simulink model "ScaraRobotApresentacao2023"  (R2024a)
(part 9 of 10)

et510 = dQ1.*dQ3.*m6.*t2.*t6.*t8.*t10.*t11.*t17.*-2.0-dQ1.*dQ3.*m6.*t3.*t6.*t7.*t10.*t11.*t17.*2.0+dQ1.*dQ2.*m6.*t2.*t6.*t8.*t10.*t11.*t20.*2.0+dQ1.*dQ2.*m6.*t3.*t6.*t7.*t10.*t11.*t20.*2.0-dQ1.*dQ6.*m6.*t2.*t6.*t8.*t9.*t11.*t17.*2.0-dQ1.*dQ6.*m6.*t3.*t6.*t7.*t9.*t11.*t17.*2.0+dQ1.*dQ3.*m6.*t2.*t6.*t8.*t10.*t11.*t20.*2.0+dQ1.*dQ3.*m6.*t3.*t6.*t7.*t10.*t11.*t20.*2.0-dQ2.*dQ3.*m6.*t4.*t6.*t9.*t10.*t11.*t17.*2.0+dQ1.*dQ6.*m6.*t2.*t6.*t8.*t9.*t11.*t20.*2.0+dQ1.*dQ6.*m6.*t3.*t6.*t7.*t9.*t11.*t20.*2.0+dQ2.*dQ3.*m6.*t4.*t6.*t9.*t10.*t11.*t20.*2.0+dQ1.*dQ4.*m6.*t2.*t3.*t5.*t10.*t17.*t36.*2.0-dQ1.*dQ4.*m6.*t2.*t3.*t5.*t10.*t20.*t36.*2.0-dQ1.*dQ6.*m6.*t2.*t4.*t5.*t8.*t20.*t36.*2.0-dQ1.*dQ6.*m6.*t3.*t4.*t5.*t7.*t20.*t36.*2.0-dQ1.*dQ4.*m6.*t5.*t7.*t8.*t10.*t17.*t36.*2.0;
et511 = dQ1.*dQ4.*m6.*t5.*t7.*t8.*t10.*t20.*t36.*2.0-dQ1.*dQ2.*m6.*t2.*t3.*t9.*t17.*t35.*t36.*2.0-dQ1.*dQ3.*m6.*t2.*t3.*t9.*t17.*t35.*t36.*2.0+dQ1.*dQ2.*m6.*t2.*t3.*t9.*t20.*t35.*t36.*2.0+dQ1.*dQ3.*m6.*t2.*t3.*t9.*t20.*t35.*t36.*2.0-dQ1.*dQ4.*m6.*t2.*t4.*t8.*t20.*t35.*t36.*2.0-dQ1.*dQ4.*m6.*t3.*t4.*t7.*t20.*t35.*t36.*2.0+dQ1.*dQ2.*m6.*t7.*t8.*t9.*t17.*t35.*t36.*2.0+dQ1.*dQ3.*m6.*t7.*t8.*t9.*t17.*t35.*t36.*2.0-dQ1.*dQ2.*m6.*t7.*t8.*t9.*t20.*t35.*t36.*2.0-dQ1.*dQ3.*m6.*t7.*t8.*t9.*t20.*t35.*t36.*2.0+Lx3.*Lxcm5.*dQ1.*dQ2.*m5.*t2.*t8.*t9.*t10.*2.0+Lx3.*Lxcm5.*dQ1.*dQ2.*m5.*t3.*t7.*t9.*t10.*2.0+Lx3.*Lxcm5.*dQ1.*dQ3.*m5.*t2.*t8.*t9.*t10.*2.0+Lx3.*Lxcm5.*dQ1.*dQ3.*m5.*t3.*t7.*t9.*t10.*2.0+Lx2.*Lxcm6.*dQ1.*dQ2.*m6.*t6.*t7.*t9.*t10.*2.0-Lx2.*Lycm6.*dQ1.*dQ2.*m6.*t7.*t9.*t10.*t11.*2.0;
et512 = Lxcm5.*Lycm5.*dQ1.*dQ4.*m5.*t2.*t5.*t8.*t9.*-2.0-Lxcm5.*Lycm5.*dQ1.*dQ4.*m5.*t3.*t5.*t7.*t9.*2.0+Lxcm6.*Lycm6.*dQ1.*dQ4.*m6.*t2.*t5.*t8.*t9.*2.0+Lxcm6.*Lycm6.*dQ1.*dQ4.*m6.*t3.*t5.*t7.*t9.*2.0+Lxcm6.*Lycm6.*dQ2.*dQ3.*m6.*t5.*t6.*t10.*t11.*4.0+Lxcm6.*Lycm6.*dQ2.*dQ6.*m6.*t5.*t6.*t9.*t11.*4.0+Lxcm6.*Lycm6.*dQ3.*dQ6.*m6.*t5.*t6.*t9.*t11.*4.0+Lxcm5.*Lycm5.*dQ1.*dQ2.*m5.*t2.*t8.*t10.*t34.*2.0+Lxcm5.*Lycm5.*dQ1.*dQ2.*m5.*t3.*t7.*t10.*t34.*2.0+Lxcm5.*Lycm5.*dQ1.*dQ3.*m5.*t2.*t8.*t10.*t34.*2.0+Lxcm5.*Lycm5.*dQ1.*dQ3.*m5.*t3.*t7.*t10.*t34.*2.0-Lxcm6.*Lycm6.*dQ1.*dQ2.*m6.*t2.*t8.*t10.*t34.*2.0-Lxcm6.*Lycm6.*dQ1.*dQ2.*m6.*t3.*t7.*t10.*t34.*2.0-Lxcm6.*Lycm6.*dQ1.*dQ3.*m6.*t2.*t8.*t10.*t34.*2.0-Lxcm6.*Lycm6.*dQ1.*dQ3.*m6.*t3.*t7.*t10.*t34.*2.0-Lxcm6.*Lycm6.*dQ1.*dQ2.*m6.*t2.*t8.*t10.*t36.*4.0-Lxcm6.*Lycm6.*dQ1.*dQ2.*m6.*t3.*t7.*t10.*t36.*4.0;
et513 = Lxcm6.*Lycm6.*dQ1.*dQ3.*m6.*t2.*t8.*t10.*t36.*-4.0-Lxcm6.*Lycm6.*dQ1.*dQ3.*m6.*t3.*t7.*t10.*t36.*4.0-Lxcm6.*Lycm6.*dQ1.*dQ6.*m6.*t2.*t8.*t9.*t36.*4.0-Lxcm6.*Lycm6.*dQ1.*dQ6.*m6.*t3.*t7.*t9.*t36.*4.0-Lxcm6.*Lycm6.*dQ2.*dQ3.*m6.*t4.*t9.*t10.*t36.*4.0+Lxcm6.*Lycm6.*dQ2.*dQ4.*m6.*t6.*t9.*t11.*t35.*4.0+Lxcm6.*Lycm6.*dQ3.*dQ4.*m6.*t6.*t9.*t11.*t35.*4.0-Lx3.*Lz5.*dQ1.*dQ2.*m6.*t2.*t5.*t8.*t9.*2.0-Lx3.*Lz5.*dQ1.*dQ2.*m6.*t3.*t5.*t7.*t9.*2.0-Lx3.*Lz5.*dQ1.*dQ3.*m6.*t2.*t5.*t8.*t9.*2.0-Lx3.*Lz5.*dQ1.*dQ3.*m6.*t3.*t5.*t7.*t9.*2.0-Lx3.*Lzcm5.*dQ1.*dQ2.*m5.*t2.*t5.*t8.*t9.*2.0-Lx3.*Lzcm5.*dQ1.*dQ2.*m5.*t3.*t5.*t7.*t9.*2.0-Lxcm6.*Lz5.*dQ1.*dQ6.*m6.*t2.*t3.*t5.*t6.*2.0-Lx3.*Lzcm5.*dQ1.*dQ3.*m5.*t2.*t5.*t8.*t9.*2.0-Lx3.*Lzcm5.*dQ1.*dQ3.*m5.*t3.*t5.*t7.*t9.*2.0;
et514 = Lxcm5.*Lz4.*dQ1.*dQ2.*m5.*t2.*t3.*t9.*t10.*-2.0-Lx3.*Lzcm6.*dQ1.*dQ2.*m6.*t2.*t5.*t8.*t9.*2.0-Lx3.*Lzcm6.*dQ1.*dQ2.*m6.*t3.*t5.*t7.*t9.*2.0-Lxcm5.*Lz4.*dQ1.*dQ3.*m5.*t2.*t3.*t9.*t10.*2.0-Lx3.*Lzcm6.*dQ1.*dQ3.*m6.*t2.*t5.*t8.*t9.*2.0-Lx3.*Lzcm6.*dQ1.*dQ3.*m6.*t3.*t5.*t7.*t9.*2.0+Lxcm6.*Lz5.*dQ1.*dQ2.*m6.*t2.*t5.*t8.*t11.*2.0+Lxcm6.*Lz5.*dQ1.*dQ2.*m6.*t3.*t5.*t7.*t11.*2.0+Lxcm6.*Lz5.*dQ1.*dQ3.*m6.*t2.*t5.*t8.*t11.*2.0+Lxcm6.*Lz5.*dQ1.*dQ3.*m6.*t3.*t5.*t7.*t11.*2.0+Lxcm6.*Lz5.*dQ1.*dQ6.*m6.*t5.*t6.*t7.*t8.*2.0+Lxcm5.*Lz4.*dQ1.*dQ2.*m5.*t7.*t8.*t9.*t10.*2.0+Lxcm6.*Lz5.*dQ2.*dQ3.*m6.*t4.*t5.*t9.*t11.*2.0+Lxcm5.*Lz4.*dQ1.*dQ3.*m5.*t7.*t8.*t9.*t10.*2.0-Lxcm6.*Lz5.*dQ2.*dQ4.*m6.*t5.*t6.*t9.*t10.*4.0-Lxcm6.*Lz5.*dQ3.*dQ4.*m6.*t5.*t6.*t9.*t10.*4.0-Lxcm6.*Lz5.*dQ1.*dQ4.*m6.*t2.*t3.*t6.*t35.*4.0;
et515 = Lxcm6.*Lz5.*dQ1.*dQ4.*m6.*t6.*t7.*t8.*t35.*4.0+Lxcm5.*Lzcm5.*dQ1.*dQ2.*m5.*t2.*t4.*t8.*t9.*2.0+Lxcm5.*Lzcm5.*dQ1.*dQ2.*m5.*t3.*t4.*t7.*t9.*2.0-Lxcm6.*Lzcm6.*dQ1.*dQ6.*m6.*t2.*t3.*t5.*t6.*2.0+Lxcm5.*Lzcm5.*dQ1.*dQ3.*m5.*t2.*t4.*t8.*t9.*2.0+Lxcm5.*Lzcm5.*dQ1.*dQ3.*m5.*t3.*t4.*t7.*t9.*2.0+Lxcm6.*Lzcm6.*dQ1.*dQ2.*m6.*t2.*t5.*t8.*t11.*2.0+Lxcm6.*Lzcm6.*dQ1.*dQ2.*m6.*t3.*t5.*t7.*t11.*2.0+Lxcm6.*Lzcm6.*dQ1.*dQ3.*m6.*t2.*t5.*t8.*t11.*2.0+Lxcm6.*Lzcm6.*dQ1.*dQ3.*m6.*t3.*t5.*t7.*t11.*2.0+Lxcm6.*Lzcm6.*dQ1.*dQ6.*m6.*t5.*t6.*t7.*t8.*2.0+Lxcm6.*Lzcm6.*dQ2.*dQ3.*m6.*t4.*t5.*t9.*t11.*2.0-Lxcm6.*Lzcm6.*dQ2.*dQ4.*m6.*t5.*t6.*t9.*t10.*4.0-Lxcm6.*Lzcm6.*dQ3.*dQ4.*m6.*t5.*t6.*t9.*t10.*4.0-Lxcm6.*Lzcm6.*dQ1.*dQ4.*m6.*t2.*t3.*t6.*t35.*4.0+Lxcm6.*Lzcm6.*dQ1.*dQ4.*m6.*t6.*t7.*t8.*t35.*4.0+Lycm6.*Lz5.*dQ1.*dQ2.*m6.*t2.*t5.*t6.*t8.*2.0;
et516 = Lycm6.*Lz5.*dQ1.*dQ2.*m6.*t3.*t5.*t6.*t7.*2.0+Lycm6.*Lz5.*dQ1.*dQ3.*m6.*t2.*t5.*t6.*t8.*2.0+Lycm6.*Lz5.*dQ1.*dQ3.*m6.*t3.*t5.*t6.*t7.*2.0+Lycm6.*Lz5.*dQ1.*dQ6.*m6.*t2.*t3.*t5.*t11.*2.0+Lycm6.*Lz5.*dQ2.*dQ3.*m6.*t4.*t5.*t6.*t9.*2.0-Lycm6.*Lz5.*dQ1.*dQ6.*m6.*t5.*t7.*t8.*t11.*2.0+Lycm6.*Lz5.*dQ2.*dQ4.*m6.*t5.*t9.*t10.*t11.*4.0+Lycm6.*Lz5.*dQ3.*dQ4.*m6.*t5.*t9.*t10.*t11.*4.0+Lycm6.*Lz5.*dQ1.*dQ4.*m6.*t2.*t3.*t11.*t35.*4.0-Lycm6.*Lz5.*dQ1.*dQ4.*m6.*t7.*t8.*t11.*t35.*4.0+Lycm6.*Lzcm6.*dQ1.*dQ2.*m6.*t2.*t5.*t6.*t8.*2.0+Lycm6.*Lzcm6.*dQ1.*dQ2.*m6.*t3.*t5.*t6.*t7.*2.0+Lycm6.*Lzcm6.*dQ1.*dQ3.*m6.*t2.*t5.*t6.*t8.*2.0+Lycm6.*Lzcm6.*dQ1.*dQ3.*m6.*t3.*t5.*t6.*t7.*2.0+Lycm6.*Lzcm6.*dQ1.*dQ6.*m6.*t2.*t3.*t5.*t11.*2.0+Lycm6.*Lzcm6.*dQ2.*dQ3.*m6.*t4.*t5.*t6.*t9.*2.0-Lycm5.*Lzcm5.*dQ1.*dQ4.*m5.*t2.*t8.*t9.*t10.*2.0;
et517 = Lycm5.*Lzcm5.*dQ1.*dQ4.*m5.*t3.*t7.*t9.*t10.*-2.0-Lycm6.*Lzcm6.*dQ1.*dQ6.*m6.*t5.*t7.*t8.*t11.*2.0+Lycm6.*Lzcm6.*dQ2.*dQ4.*m6.*t5.*t9.*t10.*t11.*4.0+Lycm6.*Lzcm6.*dQ3.*dQ4.*m6.*t5.*t9.*t10.*t11.*4.0-Lycm5.*Lzcm5.*dQ1.*dQ2.*m5.*t2.*t5.*t8.*t34.*2.0-Lycm5.*Lzcm5.*dQ1.*dQ2.*m5.*t3.*t5.*t7.*t34.*2.0-Lycm5.*Lzcm5.*dQ1.*dQ3.*m5.*t2.*t5.*t8.*t34.*2.0-Lycm5.*Lzcm5.*dQ1.*dQ3.*m5.*t3.*t5.*t7.*t34.*2.0+Lycm6.*Lzcm6.*dQ1.*dQ4.*m6.*t2.*t3.*t11.*t35.*4.0-Lycm6.*Lzcm6.*dQ1.*dQ4.*m6.*t7.*t8.*t11.*t35.*4.0+Lz4.*Lz5.*dQ1.*dQ2.*m6.*t2.*t3.*t5.*t9.*2.0+Lz4.*Lz5.*dQ1.*dQ3.*m6.*t2.*t3.*t5.*t9.*2.0-Lz4.*Lz5.*dQ1.*dQ2.*m6.*t5.*t7.*t8.*t9.*2.0-Lz4.*Lz5.*dQ1.*dQ3.*m6.*t5.*t7.*t8.*t9.*2.0+Lz4.*Lzcm5.*dQ1.*dQ2.*m5.*t2.*t3.*t5.*t9.*2.0+Lz4.*Lzcm5.*dQ1.*dQ3.*m5.*t2.*t3.*t5.*t9.*2.0+Lz4.*Lzcm6.*dQ1.*dQ2.*m6.*t2.*t3.*t5.*t9.*2.0;
et518 = Lz4.*Lzcm6.*dQ1.*dQ3.*m6.*t2.*t3.*t5.*t9.*2.0-Lz5.*Lzcm6.*dQ1.*dQ4.*m6.*t2.*t3.*t5.*t10.*4.0-Lz4.*Lzcm5.*dQ1.*dQ2.*m5.*t5.*t7.*t8.*t9.*2.0-Lz4.*Lzcm5.*dQ1.*dQ3.*m5.*t5.*t7.*t8.*t9.*2.0-Lz4.*Lzcm6.*dQ1.*dQ2.*m6.*t5.*t7.*t8.*t9.*2.0-Lz4.*Lzcm6.*dQ1.*dQ3.*m6.*t5.*t7.*t8.*t9.*2.0+Lz5.*Lzcm6.*dQ1.*dQ4.*m6.*t5.*t7.*t8.*t10.*4.0+Lz5.*Lzcm6.*dQ1.*dQ2.*m6.*t2.*t3.*t9.*t35.*4.0+Lz5.*Lzcm6.*dQ1.*dQ3.*m6.*t2.*t3.*t9.*t35.*4.0-Lz5.*Lzcm6.*dQ1.*dQ4.*m6.*t2.*t4.*t8.*t35.*4.0-Lz5.*Lzcm6.*dQ1.*dQ4.*m6.*t3.*t4.*t7.*t35.*4.0-Lz5.*Lzcm6.*dQ1.*dQ2.*m6.*t7.*t8.*t9.*t35.*4.0-Lz5.*Lzcm6.*dQ1.*dQ3.*m6.*t7.*t8.*t9.*t35.*4.0+Lx3.*Lxcm6.*dQ1.*dQ2.*m6.*t2.*t6.*t8.*t9.*t10.*2.0+Lx3.*Lxcm6.*dQ1.*dQ2.*m6.*t3.*t6.*t7.*t9.*t10.*2.0+Lx3.*Lxcm6.*dQ1.*dQ3.*m6.*t2.*t6.*t8.*t9.*t10.*2.0+Lx3.*Lxcm6.*dQ1.*dQ3.*m6.*t3.*t6.*t7.*t9.*t10.*2.0;
et519 = Lx3.*Lycm6.*dQ1.*dQ2.*m6.*t2.*t8.*t9.*t10.*t11.*-2.0-Lx3.*Lycm6.*dQ1.*dQ2.*m6.*t3.*t7.*t9.*t10.*t11.*2.0-Lx3.*Lycm6.*dQ1.*dQ3.*m6.*t2.*t8.*t9.*t10.*t11.*2.0-Lx3.*Lycm6.*dQ1.*dQ3.*m6.*t3.*t7.*t9.*t10.*t11.*2.0-Lxcm6.*Lycm6.*dQ1.*dQ2.*m6.*t2.*t3.*t6.*t9.*t11.*4.0-Lxcm6.*Lycm6.*dQ1.*dQ3.*m6.*t2.*t3.*t6.*t9.*t11.*4.0-Lxcm6.*Lycm6.*dQ1.*dQ6.*m6.*t2.*t3.*t6.*t10.*t11.*4.0+Lxcm6.*Lycm6.*dQ1.*dQ2.*m6.*t6.*t7.*t8.*t9.*t11.*4.0+Lxcm6.*Lycm6.*dQ1.*dQ3.*m6.*t6.*t7.*t8.*t9.*t11.*4.0+Lxcm6.*Lycm6.*dQ1.*dQ6.*m6.*t6.*t7.*t8.*t10.*t11.*4.0-Lxcm6.*Lycm6.*dQ1.*dQ4.*m6.*t2.*t5.*t8.*t9.*t36.*4.0-Lxcm6.*Lycm6.*dQ1.*dQ4.*m6.*t3.*t5.*t7.*t9.*t36.*4.0-Lxcm6.*Lycm6.*dQ2.*dQ3.*m6.*t5.*t6.*t10.*t11.*t34.*4.0+Lxcm6.*Lycm6.*dQ1.*dQ2.*m6.*t2.*t8.*t10.*t34.*t36.*4.0+Lxcm6.*Lycm6.*dQ1.*dQ2.*m6.*t3.*t7.*t10.*t34.*t36.*4.0;
et520 = Lxcm6.*Lycm6.*dQ1.*dQ3.*m6.*t2.*t8.*t10.*t34.*t36.*4.0+Lxcm6.*Lycm6.*dQ1.*dQ3.*m6.*t3.*t7.*t10.*t34.*t36.*4.0-Lxcm6.*Lz4.*dQ1.*dQ2.*m6.*t2.*t3.*t6.*t9.*t10.*2.0+Lxcm6.*Lz5.*dQ1.*dQ2.*m6.*t2.*t4.*t6.*t8.*t9.*2.0+Lxcm6.*Lz5.*dQ1.*dQ2.*m6.*t3.*t4.*t6.*t7.*t9.*2.0-Lxcm6.*Lz4.*dQ1.*dQ3.*m6.*t2.*t3.*t6.*t9.*t10.*2.0+Lxcm6.*Lz5.*dQ1.*dQ3.*m6.*t2.*t4.*t6.*t8.*t9.*2.0+Lxcm6.*Lz5.*dQ1.*dQ3.*m6.*t3.*t4.*t6.*t7.*t9.*2.0+Lxcm6.*Lz5.*dQ1.*dQ6.*m6.*t2.*t4.*t6.*t8.*t10.*2.0+Lxcm6.*Lz5.*dQ1.*dQ6.*m6.*t3.*t4.*t6.*t7.*t10.*2.0+Lxcm6.*Lz4.*dQ1.*dQ2.*m6.*t6.*t7.*t8.*t9.*t10.*2.0+Lxcm6.*Lz4.*dQ1.*dQ3.*m6.*t6.*t7.*t8.*t9.*t10.*2.0-Lxcm6.*Lz5.*dQ1.*dQ4.*m6.*t2.*t8.*t9.*t10.*t11.*2.0-Lxcm6.*Lz5.*dQ1.*dQ4.*m6.*t3.*t7.*t9.*t10.*t11.*2.0-Lxcm6.*Lz5.*dQ1.*dQ2.*m6.*t2.*t5.*t8.*t11.*t34.*2.0-Lxcm6.*Lz5.*dQ1.*dQ2.*m6.*t3.*t5.*t7.*t11.*t34.*2.0;
et521 = Lxcm6.*Lz5.*dQ1.*dQ3.*m6.*t2.*t5.*t8.*t11.*t34.*-2.0-Lxcm6.*Lz5.*dQ1.*dQ3.*m6.*t3.*t5.*t7.*t11.*t34.*2.0-Lxcm5.*Lzcm5.*dQ1.*dQ2.*m5.*t2.*t3.*t5.*t9.*t10.*4.0-Lxcm5.*Lzcm5.*dQ1.*dQ3.*m5.*t2.*t3.*t5.*t9.*t10.*4.0+Lxcm5.*Lzcm5.*dQ1.*dQ4.*m5.*t2.*t4.*t5.*t8.*t10.*4.0+Lxcm5.*Lzcm5.*dQ1.*dQ4.*m5.*t3.*t4.*t5.*t7.*t10.*4.0+Lxcm6.*Lzcm6.*dQ1.*dQ2.*m6.*t2.*t4.*t6.*t8.*t9.*2.0+Lxcm6.*Lzcm6.*dQ1.*dQ2.*m6.*t3.*t4.*t6.*t7.*t9.*2.0+Lxcm6.*Lzcm6.*dQ1.*dQ3.*m6.*t2.*t4.*t6.*t8.*t9.*2.0+Lxcm6.*Lzcm6.*dQ1.*dQ3.*m6.*t3.*t4.*t6.*t7.*t9.*2.0+Lxcm6.*Lzcm6.*dQ1.*dQ6.*m6.*t2.*t4.*t6.*t8.*t10.*2.0+Lxcm6.*Lzcm6.*dQ1.*dQ6.*m6.*t3.*t4.*t6.*t7.*t10.*2.0+Lxcm5.*Lzcm5.*dQ1.*dQ2.*m5.*t5.*t7.*t8.*t9.*t10.*4.0+Lxcm5.*Lzcm5.*dQ1.*dQ3.*m5.*t5.*t7.*t8.*t9.*t10.*4.0-Lxcm6.*Lzcm6.*dQ1.*dQ4.*m6.*t2.*t8.*t9.*t10.*t11.*2.0-Lxcm6.*Lzcm6.*dQ1.*dQ4.*m6.*t3.*t7.*t9.*t10.*t11.*2.0;
et522 = Lxcm5.*Lzcm5.*dQ1.*dQ2.*m5.*t2.*t4.*t8.*t9.*t35.*-4.0-Lxcm5.*Lzcm5.*dQ1.*dQ2.*m5.*t3.*t4.*t7.*t9.*t35.*4.0-Lxcm5.*Lzcm5.*dQ1.*dQ3.*m5.*t2.*t4.*t8.*t9.*t35.*4.0-Lxcm5.*Lzcm5.*dQ1.*dQ3.*m5.*t3.*t4.*t7.*t9.*t35.*4.0-Lxcm6.*Lzcm6.*dQ1.*dQ2.*m6.*t2.*t5.*t8.*t11.*t34.*2.0-Lxcm6.*Lzcm6.*dQ1.*dQ2.*m6.*t3.*t5.*t7.*t11.*t34.*2.0-Lxcm6.*Lzcm6.*dQ1.*dQ3.*m6.*t2.*t5.*t8.*t11.*t34.*2.0-Lxcm6.*Lzcm6.*dQ1.*dQ3.*m6.*t3.*t5.*t7.*t11.*t34.*2.0+Lycm6.*Lz4.*dQ1.*dQ2.*m6.*t2.*t3.*t9.*t10.*t11.*2.0-Lycm6.*Lz5.*dQ1.*dQ2.*m6.*t2.*t4.*t8.*t9.*t11.*2.0-Lycm6.*Lz5.*dQ1.*dQ2.*m6.*t3.*t4.*t7.*t9.*t11.*2.0+Lycm6.*Lz4.*dQ1.*dQ3.*m6.*t2.*t3.*t9.*t10.*t11.*2.0-Lycm6.*Lz5.*dQ1.*dQ3.*m6.*t2.*t4.*t8.*t9.*t11.*2.0-Lycm6.*Lz5.*dQ1.*dQ3.*m6.*t3.*t4.*t7.*t9.*t11.*2.0-Lycm6.*Lz5.*dQ1.*dQ4.*m6.*t2.*t6.*t8.*t9.*t10.*2.0;
et523 = Lycm6.*Lz5.*dQ1.*dQ4.*m6.*t3.*t6.*t7.*t9.*t10.*-2.0-Lycm6.*Lz5.*dQ1.*dQ6.*m6.*t2.*t4.*t8.*t10.*t11.*2.0-Lycm6.*Lz5.*dQ1.*dQ6.*m6.*t3.*t4.*t7.*t10.*t11.*2.0-Lycm6.*Lz4.*dQ1.*dQ2.*m6.*t7.*t8.*t9.*t10.*t11.*2.0-Lycm6.*Lz4.*dQ1.*dQ3.*m6.*t7.*t8.*t9.*t10.*t11.*2.0-Lycm6.*Lz5.*dQ1.*dQ2.*m6.*t2.*t5.*t6.*t8.*t34.*2.0-Lycm6.*Lz5.*dQ1.*dQ2.*m6.*t3.*t5.*t6.*t7.*t34.*2.0-Lycm6.*Lz5.*dQ1.*dQ3.*m6.*t2.*t5.*t6.*t8.*t34.*2.0-Lycm6.*Lz5.*dQ1.*dQ3.*m6.*t3.*t5.*t6.*t7.*t34.*2.0-Lycm6.*Lzcm6.*dQ1.*dQ2.*m6.*t2.*t4.*t8.*t9.*t11.*2.0-Lycm6.*Lzcm6.*dQ1.*dQ2.*m6.*t3.*t4.*t7.*t9.*t11.*2.0-Lycm6.*Lzcm6.*dQ1.*dQ3.*m6.*t2.*t4.*t8.*t9.*t11.*2.0-Lycm6.*Lzcm6.*dQ1.*dQ3.*m6.*t3.*t4.*t7.*t9.*t11.*2.0-Lycm6.*Lzcm6.*dQ1.*dQ4.*m6.*t2.*t6.*t8.*t9.*t10.*2.0-Lycm6.*Lzcm6.*dQ1.*dQ4.*m6.*t3.*t6.*t7.*t9.*t10.*2.0;
et524 = Lycm6.*Lzcm6.*dQ1.*dQ6.*m6.*t2.*t4.*t8.*t10.*t11.*-2.0-Lycm6.*Lzcm6.*dQ1.*dQ6.*m6.*t3.*t4.*t7.*t10.*t11.*2.0-Lycm6.*Lzcm6.*dQ1.*dQ2.*m6.*t2.*t5.*t6.*t8.*t34.*2.0-Lycm6.*Lzcm6.*dQ1.*dQ2.*m6.*t3.*t5.*t6.*t7.*t34.*2.0-Lycm6.*Lzcm6.*dQ1.*dQ3.*m6.*t2.*t5.*t6.*t8.*t34.*2.0-Lycm6.*Lzcm6.*dQ1.*dQ3.*m6.*t3.*t5.*t6.*t7.*t34.*2.0-Ixx6.*dQ1.*dQ2.*t2.*t4.*t5.*t8.*t9.*t10.*t36.*2.0-Ixx6.*dQ1.*dQ2.*t3.*t4.*t5.*t7.*t9.*t10.*t36.*2.0-Ixx6.*dQ1.*dQ3.*t2.*t4.*t5.*t8.*t9.*t10.*t36.*2.0-Ixx6.*dQ1.*dQ3.*t3.*t4.*t5.*t7.*t9.*t10.*t36.*2.0+Iyy6.*dQ1.*dQ2.*t2.*t4.*t5.*t8.*t9.*t10.*t36.*2.0+Iyy6.*dQ1.*dQ2.*t3.*t4.*t5.*t7.*t9.*t10.*t36.*2.0+Iyy6.*dQ1.*dQ3.*t2.*t4.*t5.*t8.*t9.*t10.*t36.*2.0+Iyy6.*dQ1.*dQ3.*t3.*t4.*t5.*t7.*t9.*t10.*t36.*2.0+dQ1.*dQ2.*m5.*t2.*t4.*t5.*t8.*t9.*t10.*t16.*2.0;
et525 = dQ1.*dQ2.*m5.*t3.*t4.*t5.*t7.*t9.*t10.*t16.*2.0+dQ1.*dQ3.*m5.*t2.*t4.*t5.*t8.*t9.*t10.*t16.*2.0+dQ1.*dQ3.*m5.*t3.*t4.*t5.*t7.*t9.*t10.*t16.*2.0+dQ1.*dQ2.*m6.*t2.*t4.*t5.*t8.*t9.*t10.*t20.*2.0+dQ1.*dQ2.*m6.*t3.*t4.*t5.*t7.*t9.*t10.*t20.*2.0+dQ1.*dQ3.*m6.*t2.*t4.*t5.*t8.*t9.*t10.*t20.*2.0+dQ1.*dQ3.*m6.*t3.*t4.*t5.*t7.*t9.*t10.*t20.*2.0-dQ1.*dQ2.*m6.*t2.*t4.*t5.*t8.*t9.*t10.*t22.*2.0-dQ1.*dQ2.*m6.*t3.*t4.*t5.*t7.*t9.*t10.*t22.*2.0-dQ1.*dQ4.*m6.*t2.*t5.*t6.*t8.*t9.*t11.*t17.*2.0-dQ1.*dQ4.*m6.*t3.*t5.*t6.*t7.*t9.*t11.*t17.*2.0-dQ1.*dQ3.*m6.*t2.*t4.*t5.*t8.*t9.*t10.*t22.*2.0-dQ1.*dQ3.*m6.*t3.*t4.*t5.*t7.*t9.*t10.*t22.*2.0-dQ1.*dQ2.*m5.*t2.*t4.*t5.*t8.*t9.*t10.*t25.*2.0-dQ1.*dQ2.*m5.*t3.*t4.*t5.*t7.*t9.*t10.*t25.*2.0;
et526 = dQ1.*dQ3.*m5.*t2.*t4.*t5.*t8.*t9.*t10.*t25.*-2.0-dQ1.*dQ3.*m5.*t3.*t4.*t5.*t7.*t9.*t10.*t25.*2.0+dQ1.*dQ4.*m6.*t2.*t5.*t6.*t8.*t9.*t11.*t20.*2.0+dQ1.*dQ4.*m6.*t3.*t5.*t6.*t7.*t9.*t11.*t20.*2.0-dQ1.*dQ2.*m6.*t2.*t4.*t5.*t8.*t9.*t10.*t26.*2.0-dQ1.*dQ2.*m6.*t3.*t4.*t5.*t7.*t9.*t10.*t26.*2.0-dQ1.*dQ3.*m6.*t2.*t4.*t5.*t8.*t9.*t10.*t26.*2.0-dQ1.*dQ3.*m6.*t3.*t4.*t5.*t7.*t9.*t10.*t26.*2.0+dQ1.*dQ2.*m6.*t2.*t6.*t8.*t10.*t11.*t17.*t34.*2.0+dQ1.*dQ2.*m6.*t3.*t6.*t7.*t10.*t11.*t17.*t34.*2.0+dQ1.*dQ3.*m6.*t2.*t6.*t8.*t10.*t11.*t17.*t34.*2.0+dQ1.*dQ3.*m6.*t3.*t6.*t7.*t10.*t11.*t17.*t34.*2.0-dQ1.*dQ2.*m6.*t2.*t6.*t8.*t10.*t11.*t20.*t34.*2.0-dQ1.*dQ2.*m6.*t3.*t6.*t7.*t10.*t11.*t20.*t34.*2.0-dQ1.*dQ3.*m6.*t2.*t6.*t8.*t10.*t11.*t20.*t34.*2.0;
et527 = dQ1.*dQ3.*m6.*t3.*t6.*t7.*t10.*t11.*t20.*t34.*-2.0-Ixy6.*dQ1.*dQ2.*t2.*t4.*t5.*t6.*t8.*t9.*t10.*t11.*2.0-Ixy6.*dQ1.*dQ2.*t3.*t4.*t5.*t6.*t7.*t9.*t10.*t11.*2.0-Ixy6.*dQ1.*dQ3.*t2.*t4.*t5.*t6.*t8.*t9.*t10.*t11.*2.0-Ixy6.*dQ1.*dQ3.*t3.*t4.*t5.*t6.*t7.*t9.*t10.*t11.*2.0-Iyx6.*dQ1.*dQ2.*t2.*t4.*t5.*t6.*t8.*t9.*t10.*t11.*2.0-Iyx6.*dQ1.*dQ2.*t3.*t4.*t5.*t6.*t7.*t9.*t10.*t11.*2.0-Iyx6.*dQ1.*dQ3.*t2.*t4.*t5.*t6.*t8.*t9.*t10.*t11.*2.0-Iyx6.*dQ1.*dQ3.*t3.*t4.*t5.*t6.*t7.*t9.*t10.*t11.*2.0+dQ1.*dQ2.*m6.*t2.*t4.*t5.*t8.*t9.*t10.*t17.*t36.*2.0+dQ1.*dQ2.*m6.*t3.*t4.*t5.*t7.*t9.*t10.*t17.*t36.*2.0+dQ1.*dQ3.*m6.*t2.*t4.*t5.*t8.*t9.*t10.*t17.*t36.*2.0+dQ1.*dQ3.*m6.*t3.*t4.*t5.*t7.*t9.*t10.*t17.*t36.*2.0-dQ1.*dQ2.*m6.*t2.*t4.*t5.*t8.*t9.*t10.*t20.*t36.*2.0;
et528 = dQ1.*dQ2.*m6.*t3.*t4.*t5.*t7.*t9.*t10.*t20.*t36.*-2.0-dQ1.*dQ3.*m6.*t2.*t4.*t5.*t8.*t9.*t10.*t20.*t36.*2.0-dQ1.*dQ3.*m6.*t3.*t4.*t5.*t7.*t9.*t10.*t20.*t36.*2.0-Lxcm6.*Lycm6.*dQ1.*dQ4.*m6.*t2.*t3.*t5.*t6.*t10.*t11.*4.0-Lxcm6.*Lycm6.*dQ1.*dQ6.*m6.*t2.*t4.*t5.*t6.*t8.*t11.*4.0-Lxcm6.*Lycm6.*dQ1.*dQ6.*m6.*t3.*t4.*t5.*t6.*t7.*t11.*4.0+Lxcm6.*Lycm6.*dQ1.*dQ4.*m6.*t5.*t6.*t7.*t8.*t10.*t11.*4.0+Lxcm6.*Lycm6.*dQ1.*dQ2.*m6.*t2.*t3.*t6.*t9.*t11.*t35.*4.0+Lxcm6.*Lycm6.*dQ1.*dQ3.*m6.*t2.*t3.*t6.*t9.*t11.*t35.*4.0-Lxcm6.*Lycm6.*dQ1.*dQ4.*m6.*t2.*t4.*t6.*t8.*t11.*t35.*4.0-Lxcm6.*Lycm6.*dQ1.*dQ4.*m6.*t3.*t4.*t6.*t7.*t11.*t35.*4.0-Lxcm6.*Lycm6.*dQ1.*dQ2.*m6.*t6.*t7.*t8.*t9.*t11.*t35.*4.0-Lxcm6.*Lycm6.*dQ1.*dQ3.*m6.*t6.*t7.*t8.*t9.*t11.*t35.*4.0-Lxcm6.*Lz5.*dQ1.*dQ2.*m6.*t2.*t3.*t5.*t6.*t9.*t10.*4.0;
et529 = Lxcm6.*Lz5.*dQ1.*dQ3.*m6.*t2.*t3.*t5.*t6.*t9.*t10.*-4.0+Lxcm6.*Lz5.*dQ1.*dQ4.*m6.*t2.*t4.*t5.*t6.*t8.*t10.*4.0+Lxcm6.*Lz5.*dQ1.*dQ4.*m6.*t3.*t4.*t5.*t6.*t7.*t10.*4.0+Lxcm6.*Lz5.*dQ1.*dQ2.*m6.*t5.*t6.*t7.*t8.*t9.*t10.*4.0+Lxcm6.*Lz5.*dQ1.*dQ3.*m6.*t5.*t6.*t7.*t8.*t9.*t10.*4.0-Lxcm6.*Lz5.*dQ1.*dQ2.*m6.*t2.*t4.*t6.*t8.*t9.*t35.*4.0-Lxcm6.*Lz5.*dQ1.*dQ2.*m6.*t3.*t4.*t6.*t7.*t9.*t35.*4.0-Lxcm6.*Lz5.*dQ1.*dQ3.*m6.*t2.*t4.*t6.*t8.*t9.*t35.*4.0-Lxcm6.*Lz5.*dQ1.*dQ3.*m6.*t3.*t4.*t6.*t7.*t9.*t35.*4.0-Lxcm6.*Lzcm6.*dQ1.*dQ2.*m6.*t2.*t3.*t5.*t6.*t9.*t10.*4.0-Lxcm6.*Lzcm6.*dQ1.*dQ3.*m6.*t2.*t3.*t5.*t6.*t9.*t10.*4.0+Lxcm6.*Lzcm6.*dQ1.*dQ4.*m6.*t2.*t4.*t5.*t6.*t8.*t10.*4.0+Lxcm6.*Lzcm6.*dQ1.*dQ4.*m6.*t3.*t4.*t5.*t6.*t7.*t10.*4.0+Lxcm6.*Lzcm6.*dQ1.*dQ2.*m6.*t5.*t6.*t7.*t8.*t9.*t10.*4.0;
et530 = Lxcm6.*Lzcm6.*dQ1.*dQ3.*m6.*t5.*t6.*t7.*t8.*t9.*t10.*4.0-Lxcm6.*Lzcm6.*dQ1.*dQ2.*m6.*t2.*t4.*t6.*t8.*t9.*t35.*4.0-Lxcm6.*Lzcm6.*dQ1.*dQ2.*m6.*t3.*t4.*t6.*t7.*t9.*t35.*4.0-Lxcm6.*Lzcm6.*dQ1.*dQ3.*m6.*t2.*t4.*t6.*t8.*t9.*t35.*4.0-Lxcm6.*Lzcm6.*dQ1.*dQ3.*m6.*t3.*t4.*t6.*t7.*t9.*t35.*4.0+Lycm6.*Lz5.*dQ1.*dQ2.*m6.*t2.*t3.*t5.*t9.*t10.*t11.*4.0+Lycm6.*Lz5.*dQ1.*dQ3.*m6.*t2.*t3.*t5.*t9.*t10.*t11.*4.0-Lycm6.*Lz5.*dQ1.*dQ4.*m6.*t2.*t4.*t5.*t8.*t10.*t11.*4.0-Lycm6.*Lz5.*dQ1.*dQ4.*m6.*t3.*t4.*t5.*t7.*t10.*t11.*4.0-Lycm6.*Lz5.*dQ1.*dQ2.*m6.*t5.*t7.*t8.*t9.*t10.*t11.*4.0-Lycm6.*Lz5.*dQ1.*dQ3.*m6.*t5.*t7.*t8.*t9.*t10.*t11.*4.0+Lycm6.*Lz5.*dQ1.*dQ2.*m6.*t2.*t4.*t8.*t9.*t11.*t35.*4.0+Lycm6.*Lz5.*dQ1.*dQ2.*m6.*t3.*t4.*t7.*t9.*t11.*t35.*4.0+Lycm6.*Lz5.*dQ1.*dQ3.*m6.*t2.*t4.*t8.*t9.*t11.*t35.*4.0;
et531 = Lycm6.*Lz5.*dQ1.*dQ3.*m6.*t3.*t4.*t7.*t9.*t11.*t35.*4.0+Lycm6.*Lzcm6.*dQ1.*dQ2.*m6.*t2.*t3.*t5.*t9.*t10.*t11.*4.0+Lycm6.*Lzcm6.*dQ1.*dQ3.*m6.*t2.*t3.*t5.*t9.*t10.*t11.*4.0-Lycm6.*Lzcm6.*dQ1.*dQ4.*m6.*t2.*t4.*t5.*t8.*t10.*t11.*4.0-Lycm6.*Lzcm6.*dQ1.*dQ4.*m6.*t3.*t4.*t5.*t7.*t10.*t11.*4.0-Lycm6.*Lzcm6.*dQ1.*dQ2.*m6.*t5.*t7.*t8.*t9.*t10.*t11.*4.0-Lycm6.*Lzcm6.*dQ1.*dQ3.*m6.*t5.*t7.*t8.*t9.*t10.*t11.*4.0+Lycm6.*Lzcm6.*dQ1.*dQ2.*m6.*t2.*t4.*t8.*t9.*t11.*t35.*4.0+Lycm6.*Lzcm6.*dQ1.*dQ2.*m6.*t3.*t4.*t7.*t9.*t11.*t35.*4.0+Lycm6.*Lzcm6.*dQ1.*dQ3.*m6.*t2.*t4.*t8.*t9.*t11.*t35.*4.0+Lycm6.*Lzcm6.*dQ1.*dQ3.*m6.*t3.*t4.*t7.*t9.*t11.*t35.*4.0-Lz5.*Lzcm6.*dQ1.*dQ2.*m6.*t2.*t4.*t5.*t8.*t9.*t10.*4.0-Lz5.*Lzcm6.*dQ1.*dQ2.*m6.*t3.*t4.*t5.*t7.*t9.*t10.*4.0-Lz5.*Lzcm6.*dQ1.*dQ3.*m6.*t2.*t4.*t5.*t8.*t9.*t10.*4.0;
et532 = Lz5.*Lzcm6.*dQ1.*dQ3.*m6.*t3.*t4.*t5.*t7.*t9.*t10.*-4.0-Lxcm6.*Lycm6.*dQ1.*dQ2.*m6.*t2.*t4.*t5.*t6.*t8.*t9.*t10.*t11.*4.0-Lxcm6.*Lycm6.*dQ1.*dQ2.*m6.*t3.*t4.*t5.*t6.*t7.*t9.*t10.*t11.*4.0-Lxcm6.*Lycm6.*dQ1.*dQ3.*m6.*t2.*t4.*t5.*t6.*t8.*t9.*t10.*t11.*4.0-Lxcm6.*Lycm6.*dQ1.*dQ3.*m6.*t3.*t4.*t5.*t6.*t7.*t9.*t10.*t11.*4.0;
et533 = t9.*t10.*t55+t9.*t10.*t56+t9.*t10.*t62+t9.*t10.*t63+t9.*t10.*t82+t9.*t10.*t83+t9.*t10.*t84+t9.*t10.*t85+t9.*t10.*t88+t9.*t10.*t89+t9.*t10.*t90+t9.*t10.*t91+t9.*t10.*t138+t9.*t10.*t139+t9.*t10.*t150+t9.*t10.*t151+t9.*t10.*t177+t9.*t10.*t178+t9.*t10.*t179+t9.*t10.*t180+t9.*t10.*t307+t9.*t10.*t308+t9.*t10.*t333+t9.*t10.*t334+t9.*t10.*t342+t9.*t10.*t343+t9.*t10.*t418+t9.*t10.*t419+t9.*t10.*t615+t9.*t10.*t616+t9.*t10.*t674+t9.*t10.*t675+t9.*t10.*t687+t9.*t10.*t688+t9.*t10.*t761+t9.*t10.*t762+t9.*t10.*t776+t9.*t10.*t777+t9.*t10.*t942+t9.*t10.*t943+t9.*t10.*t1096+t9.*t10.*t1097+t9.*t10.*t1481+t9.*t10.*t1482+t9.*t10.*t1642+t9.*t10.*t1643-t9.*t10.*t36.*t138.*2.0-t9.*t10.*t36.*t139.*2.0;
et534 = -Ixx6.*dQ4.*dQ5.*t10-Ixy6.*dQ2.*dQ5.*t4-Ixy6.*dQ3.*dQ5.*t4-Ixy6.*dQ2.*dQ3.*t34+Ixy6.*dQ2.*dQ3.*t35-Iyx6.*dQ2.*dQ5.*t4-Iyx6.*dQ3.*dQ5.*t4-Iyx6.*dQ2.*dQ3.*t34+Iyx6.*dQ2.*dQ3.*t35+Iyy6.*dQ4.*dQ5.*t10-Izz6.*dQ4.*dQ5.*t10-Ixx6.*dQ2.*dQ4.*t4.*t10+Ixx6.*dQ2.*dQ5.*t5.*t9-Ixx6.*dQ3.*dQ4.*t4.*t10+Ixx6.*dQ3.*dQ5.*t5.*t9+Ixx6.*dQ4.*dQ5.*t10.*t36.*2.0+Ixy6.*dQ1.*dQ4.*t2.*t3-Ixy6.*dQ1.*dQ4.*t7.*t8+Ixy6.*dQ2.*dQ5.*t4.*t36.*2.0+Ixy6.*dQ3.*dQ5.*t4.*t36.*2.0-Ixy6.*dQ2.*dQ3.*t34.*t35+Ixy6.*dQ2.*dQ3.*t34.*t36.*2.0-Ixy6.*dQ2.*dQ3.*t35.*t36.*2.0+Ixz6.*dQ4.*dQ5.*t5.*t6+Ixz6.*dQ2.*dQ4.*t9.*t11+Ixz6.*dQ3.*dQ4.*t9.*t11+Iyx6.*dQ1.*dQ4.*t2.*t3-Iyx6.*dQ1.*dQ4.*t7.*t8+Iyx6.*dQ2.*dQ5.*t4.*t36.*2.0;
et535 = Iyx6.*dQ3.*dQ5.*t4.*t36.*2.0-Iyx6.*dQ2.*dQ3.*t34.*t35+Iyx6.*dQ2.*dQ3.*t34.*t36.*2.0-Iyx6.*dQ2.*dQ3.*t35.*t36.*2.0+Iyy6.*dQ2.*dQ4.*t4.*t10-Iyy6.*dQ2.*dQ5.*t5.*t9+Iyy6.*dQ3.*dQ4.*t4.*t10-Iyy6.*dQ3.*dQ5.*t5.*t9-Iyy6.*dQ4.*dQ5.*t10.*t36.*2.0+Iyz6.*dQ2.*dQ4.*t6.*t9+Iyz6.*dQ3.*dQ4.*t6.*t9-Iyz6.*dQ4.*dQ5.*t5.*t11+Izx6.*dQ4.*dQ5.*t5.*t6+Izx6.*dQ2.*dQ4.*t9.*t11+Izx6.*dQ3.*dQ4.*t9.*t11+Izy6.*dQ2.*dQ4.*t6.*t9+Izy6.*dQ3.*dQ4.*t6.*t9-Izy6.*dQ4.*dQ5.*t5.*t11+Izz6.*dQ2.*dQ4.*t4.*t10+Izz6.*dQ2.*dQ5.*t5.*t9+Izz6.*dQ3.*dQ4.*t4.*t10+Izz6.*dQ3.*dQ5.*t5.*t9-dQ4.*dQ5.*m6.*t10.*t20.*2.0+t4.*t5.*t6.*t10.*t11.*t130.*2.0+t4.*t5.*t6.*t10.*t11.*t131.*2.0-t4.*t5.*t6.*t10.*t11.*t138.*2.0-t4.*t5.*t6.*t10.*t11.*t139.*2.0-Lxcm6.*Lycm6.*dQ2.*dQ5.*m6.*t4.*2.0;
et536 = Lxcm6.*Lycm6.*dQ3.*dQ5.*m6.*t4.*-2.0-Lxcm6.*Lycm6.*dQ2.*dQ3.*m6.*t34.*2.0+Lxcm6.*Lycm6.*dQ2.*dQ3.*m6.*t35.*2.0+Ixx6.*dQ1.*dQ2.*t2.*t5.*t8+Ixx6.*dQ1.*dQ2.*t3.*t5.*t7+Ixx6.*dQ1.*dQ3.*t2.*t5.*t8+Ixx6.*dQ1.*dQ3.*t3.*t5.*t7-Ixx6.*dQ1.*dQ5.*t2.*t3.*t10+Ixx6.*dQ2.*dQ3.*t4.*t5.*t9.*2.0-Ixx6.*dQ2.*dQ5.*t4.*t6.*t11.*2.0-Ixx6.*dQ3.*dQ5.*t4.*t6.*t11.*2.0+Ixx6.*dQ1.*dQ5.*t7.*t8.*t10-Ixx6.*dQ2.*dQ3.*t6.*t11.*t34.*2.0+Ixx6.*dQ2.*dQ4.*t4.*t10.*t36.*2.0+Ixx6.*dQ2.*dQ3.*t6.*t11.*t35.*2.0-Ixx6.*dQ2.*dQ5.*t5.*t9.*t36.*2.0+Ixx6.*dQ3.*dQ4.*t4.*t10.*t36.*2.0-Ixx6.*dQ3.*dQ5.*t5.*t9.*t36.*2.0-Ixy6.*dQ1.*dQ5.*t2.*t8.*t9-Ixy6.*dQ1.*dQ5.*t3.*t7.*t9+Ixy6.*dQ4.*dQ5.*t6.*t10.*t11.*2.0-Ixy6.*dQ1.*dQ4.*t2.*t3.*t35-Ixy6.*dQ1.*dQ4.*t2.*t3.*t36.*2.0+Ixy6.*dQ1.*dQ4.*t7.*t8.*t35;
et537 = Ixy6.*dQ1.*dQ4.*t7.*t8.*t36.*2.0+Ixy6.*dQ2.*dQ3.*t34.*t35.*t36.*2.0-Ixz6.*dQ2.*dQ3.*t5.*t10.*t11-Ixz6.*dQ2.*dQ4.*t9.*t11.*t35-Ixz6.*dQ3.*dQ4.*t9.*t11.*t35-Iyx6.*dQ1.*dQ5.*t2.*t8.*t9-Iyx6.*dQ1.*dQ5.*t3.*t7.*t9+Iyx6.*dQ4.*dQ5.*t6.*t10.*t11.*2.0-Iyx6.*dQ1.*dQ4.*t2.*t3.*t35-Iyx6.*dQ1.*dQ4.*t2.*t3.*t36.*2.0+Iyx6.*dQ1.*dQ4.*t7.*t8.*t35+Iyx6.*dQ1.*dQ4.*t7.*t8.*t36.*2.0+Iyx6.*dQ2.*dQ3.*t34.*t35.*t36.*2.0-Iyy6.*dQ1.*dQ2.*t2.*t5.*t8-Iyy6.*dQ1.*dQ2.*t3.*t5.*t7-Iyy6.*dQ1.*dQ3.*t2.*t5.*t8-Iyy6.*dQ1.*dQ3.*t3.*t5.*t7+Iyy6.*dQ1.*dQ5.*t2.*t3.*t10-Iyy6.*dQ2.*dQ3.*t4.*t5.*t9.*2.0+Iyy6.*dQ2.*dQ5.*t4.*t6.*t11.*2.0+Iyy6.*dQ3.*dQ5.*t4.*t6.*t11.*2.0-Iyy6.*dQ1.*dQ5.*t7.*t8.*t10+Iyy6.*dQ2.*dQ3.*t6.*t11.*t34.*2.0;
et538 = Iyy6.*dQ2.*dQ4.*t4.*t10.*t36.*-2.0-Iyy6.*dQ2.*dQ3.*t6.*t11.*t35.*2.0+Iyy6.*dQ2.*dQ5.*t5.*t9.*t36.*2.0-Iyy6.*dQ3.*dQ4.*t4.*t10.*t36.*2.0+Iyy6.*dQ3.*dQ5.*t5.*t9.*t36.*2.0-Iyz6.*dQ2.*dQ3.*t5.*t6.*t10-Iyz6.*dQ2.*dQ4.*t6.*t9.*t35-Iyz6.*dQ3.*dQ4.*t6.*t9.*t35-Izx6.*dQ2.*dQ3.*t5.*t10.*t11-Izx6.*dQ2.*dQ4.*t9.*t11.*t35-Izx6.*dQ3.*dQ4.*t9.*t11.*t35-Izy6.*dQ2.*dQ3.*t5.*t6.*t10-Izy6.*dQ2.*dQ4.*t6.*t9.*t35-Izy6.*dQ3.*dQ4.*t6.*t9.*t35-Izz6.*dQ1.*dQ2.*t2.*t5.*t8-Izz6.*dQ1.*dQ2.*t3.*t5.*t7-Izz6.*dQ1.*dQ3.*t2.*t5.*t8-Izz6.*dQ1.*dQ3.*t3.*t5.*t7-Izz6.*dQ1.*dQ5.*t2.*t3.*t10+Izz6.*dQ1.*dQ5.*t7.*t8.*t10+dQ2.*dQ4.*m6.*t4.*t10.*t17.*2.0+dQ3.*dQ4.*m6.*t4.*t10.*t17.*2.0+dQ2.*dQ5.*m6.*t5.*t9.*t20.*2.0;
et539 = dQ3.*dQ5.*m6.*t5.*t9.*t20.*2.0-dQ4.*dQ5.*m6.*t10.*t17.*t36.*2.0+dQ4.*dQ5.*m6.*t10.*t20.*t36.*2.0+Lx3.*Lxcm6.*dQ2.*dQ3.*m6.*t6.*t9.*2.0-Lx3.*Lycm6.*dQ2.*dQ3.*m6.*t9.*t11.*2.0+Lxcm6.*Lycm6.*dQ1.*dQ4.*m6.*t2.*t3.*2.0-Lxcm6.*Lycm6.*dQ1.*dQ4.*m6.*t7.*t8.*2.0+Lxcm6.*Lycm6.*dQ2.*dQ5.*m6.*t4.*t36.*4.0+Lxcm6.*Lycm6.*dQ3.*dQ5.*m6.*t4.*t36.*4.0-Lxcm6.*Lycm6.*dQ2.*dQ3.*m6.*t34.*t35.*2.0+Lxcm6.*Lycm6.*dQ2.*dQ3.*m6.*t34.*t36.*4.0-Lxcm6.*Lycm6.*dQ2.*dQ3.*m6.*t35.*t36.*4.0+Lxcm6.*Lz5.*dQ4.*dQ5.*m6.*t5.*t6.*2.0-Lxcm6.*Lz4.*dQ2.*dQ3.*m6.*t10.*t11.*2.0+Lxcm6.*Lz5.*dQ2.*dQ4.*m6.*t9.*t11.*2.0+Lxcm6.*Lz5.*dQ3.*dQ4.*m6.*t9.*t11.*2.0+Lxcm6.*Lzcm6.*dQ4.*dQ5.*m6.*t5.*t6.*2.0+Lxcm6.*Lzcm6.*dQ2.*dQ4.*m6.*t9.*t11.*2.0+Lxcm6.*Lzcm6.*dQ3.*dQ4.*m6.*t9.*t11.*2.0-Lycm6.*Lz4.*dQ2.*dQ3.*m6.*t6.*t10.*2.0+Lycm6.*Lz5.*dQ2.*dQ4.*m6.*t6.*t9.*2.0;
et540 = Lycm6.*Lz5.*dQ3.*dQ4.*m6.*t6.*t9.*2.0-Lycm6.*Lz5.*dQ4.*dQ5.*m6.*t5.*t11.*2.0+Lycm6.*Lzcm6.*dQ2.*dQ4.*m6.*t6.*t9.*2.0+Lycm6.*Lzcm6.*dQ3.*dQ4.*m6.*t6.*t9.*2.0-Lycm6.*Lzcm6.*dQ4.*dQ5.*m6.*t5.*t11.*2.0-Ixx6.*dQ1.*dQ2.*t2.*t3.*t4.*t10-Ixx6.*dQ1.*dQ3.*t2.*t3.*t4.*t10-Ixx6.*dQ1.*dQ5.*t2.*t4.*t5.*t8-Ixx6.*dQ1.*dQ5.*t3.*t4.*t5.*t7+Ixx6.*dQ1.*dQ4.*t2.*t3.*t6.*t11.*2.0+Ixx6.*dQ1.*dQ2.*t4.*t7.*t8.*t10+Ixx6.*dQ1.*dQ3.*t4.*t7.*t8.*t10-Ixx6.*dQ1.*dQ4.*t6.*t7.*t8.*t11.*2.0-Ixx6.*dQ1.*dQ2.*t2.*t5.*t8.*t34.*2.0-Ixx6.*dQ1.*dQ2.*t3.*t5.*t7.*t34.*2.0-Ixx6.*dQ1.*dQ3.*t2.*t5.*t8.*t34.*2.0-Ixx6.*dQ1.*dQ3.*t3.*t5.*t7.*t34.*2.0-Ixx6.*dQ1.*dQ2.*t2.*t5.*t8.*t36.*2.0-Ixx6.*dQ1.*dQ2.*t3.*t5.*t7.*t36.*2.0-Ixx6.*dQ1.*dQ3.*t2.*t5.*t8.*t36.*2.0;
et541 = Ixx6.*dQ1.*dQ3.*t3.*t5.*t7.*t36.*-2.0+Ixx6.*dQ1.*dQ5.*t2.*t3.*t10.*t36.*2.0-Ixx6.*dQ2.*dQ3.*t4.*t5.*t9.*t36.*4.0-Ixx6.*dQ1.*dQ5.*t7.*t8.*t10.*t36.*2.0-Ixx6.*dQ2.*dQ3.*t6.*t11.*t34.*t35.*2.0-Ixy6.*dQ1.*dQ2.*t2.*t4.*t8.*t9-Ixy6.*dQ1.*dQ2.*t3.*t4.*t7.*t9-Ixy6.*dQ1.*dQ3.*t2.*t4.*t8.*t9-Ixy6.*dQ1.*dQ3.*t3.*t4.*t7.*t9+Ixy6.*dQ2.*dQ4.*t4.*t6.*t10.*t11.*2.0-Ixy6.*dQ2.*dQ5.*t5.*t6.*t9.*t11.*2.0+Ixy6.*dQ3.*dQ4.*t4.*t6.*t10.*t11.*2.0-Ixy6.*dQ3.*dQ5.*t5.*t6.*t9.*t11.*2.0+Ixy6.*dQ1.*dQ5.*t2.*t8.*t9.*t36.*2.0+Ixy6.*dQ1.*dQ5.*t3.*t7.*t9.*t36.*2.0+Ixy6.*dQ1.*dQ4.*t2.*t3.*t35.*t36.*2.0-Ixy6.*dQ1.*dQ4.*t7.*t8.*t35.*t36.*2.0+Ixz6.*dQ1.*dQ5.*t2.*t3.*t5.*t6-Ixz6.*dQ1.*dQ4.*t2.*t4.*t8.*t11-Ixz6.*dQ1.*dQ4.*t3.*t4.*t7.*t11;
et542 = -Ixz6.*dQ1.*dQ5.*t5.*t6.*t7.*t8+Ixz6.*dQ2.*dQ3.*t4.*t6.*t9.*t10+Ixz6.*dQ2.*dQ3.*t5.*t10.*t11.*t34-Iyx6.*dQ1.*dQ2.*t2.*t4.*t8.*t9-Iyx6.*dQ1.*dQ2.*t3.*t4.*t7.*t9-Iyx6.*dQ1.*dQ3.*t2.*t4.*t8.*t9-Iyx6.*dQ1.*dQ3.*t3.*t4.*t7.*t9+Iyx6.*dQ2.*dQ4.*t4.*t6.*t10.*t11.*2.0-Iyx6.*dQ2.*dQ5.*t5.*t6.*t9.*t11.*2.0+Iyx6.*dQ3.*dQ4.*t4.*t6.*t10.*t11.*2.0-Iyx6.*dQ3.*dQ5.*t5.*t6.*t9.*t11.*2.0+Iyx6.*dQ1.*dQ5.*t2.*t8.*t9.*t36.*2.0+Iyx6.*dQ1.*dQ5.*t3.*t7.*t9.*t36.*2.0+Iyx6.*dQ1.*dQ4.*t2.*t3.*t35.*t36.*2.0-Iyx6.*dQ1.*dQ4.*t7.*t8.*t35.*t36.*2.0+Iyy6.*dQ1.*dQ2.*t2.*t3.*t4.*t10+Iyy6.*dQ1.*dQ3.*t2.*t3.*t4.*t10+Iyy6.*dQ1.*dQ5.*t2.*t4.*t5.*t8+Iyy6.*dQ1.*dQ5.*t3.*t4.*t5.*t7-Iyy6.*dQ1.*dQ4.*t2.*t3.*t6.*t11.*2.0-Iyy6.*dQ1.*dQ2.*t4.*t7.*t8.*t10;
et543 = -Iyy6.*dQ1.*dQ3.*t4.*t7.*t8.*t10+Iyy6.*dQ1.*dQ4.*t6.*t7.*t8.*t11.*2.0+Iyy6.*dQ1.*dQ2.*t2.*t5.*t8.*t34.*2.0+Iyy6.*dQ1.*dQ2.*t3.*t5.*t7.*t34.*2.0+Iyy6.*dQ1.*dQ3.*t2.*t5.*t8.*t34.*2.0+Iyy6.*dQ1.*dQ3.*t3.*t5.*t7.*t34.*2.0+Iyy6.*dQ1.*dQ2.*t2.*t5.*t8.*t36.*2.0+Iyy6.*dQ1.*dQ2.*t3.*t5.*t7.*t36.*2.0+Iyy6.*dQ1.*dQ3.*t2.*t5.*t8.*t36.*2.0+Iyy6.*dQ1.*dQ3.*t3.*t5.*t7.*t36.*2.0-Iyy6.*dQ1.*dQ5.*t2.*t3.*t10.*t36.*2.0+Iyy6.*dQ2.*dQ3.*t4.*t5.*t9.*t36.*4.0+Iyy6.*dQ1.*dQ5.*t7.*t8.*t10.*t36.*2.0+Iyy6.*dQ2.*dQ3.*t6.*t11.*t34.*t35.*2.0-Iyz6.*dQ1.*dQ4.*t2.*t4.*t6.*t8-Iyz6.*dQ1.*dQ4.*t3.*t4.*t6.*t7-Iyz6.*dQ1.*dQ5.*t2.*t3.*t5.*t11+Iyz6.*dQ1.*dQ5.*t5.*t7.*t8.*t11-Iyz6.*dQ2.*dQ3.*t4.*t9.*t10.*t11+Iyz6.*dQ2.*dQ3.*t5.*t6.*t10.*t34+Izx6.*dQ1.*dQ5.*t2.*t3.*t5.*t6;
et544 = -Izx6.*dQ1.*dQ4.*t2.*t4.*t8.*t11-Izx6.*dQ1.*dQ4.*t3.*t4.*t7.*t11-Izx6.*dQ1.*dQ5.*t5.*t6.*t7.*t8+Izx6.*dQ2.*dQ3.*t4.*t6.*t9.*t10+Izx6.*dQ2.*dQ3.*t5.*t10.*t11.*t34-Izy6.*dQ1.*dQ4.*t2.*t4.*t6.*t8-Izy6.*dQ1.*dQ4.*t3.*t4.*t6.*t7-Izy6.*dQ1.*dQ5.*t2.*t3.*t5.*t11+Izy6.*dQ1.*dQ5.*t5.*t7.*t8.*t11-Izy6.*dQ2.*dQ3.*t4.*t9.*t10.*t11+Izy6.*dQ2.*dQ3.*t5.*t6.*t10.*t34-Izz6.*dQ1.*dQ2.*t2.*t3.*t4.*t10-Izz6.*dQ1.*dQ3.*t2.*t3.*t4.*t10-Izz6.*dQ1.*dQ5.*t2.*t4.*t5.*t8-Izz6.*dQ1.*dQ5.*t3.*t4.*t5.*t7+Izz6.*dQ1.*dQ2.*t4.*t7.*t8.*t10+Izz6.*dQ1.*dQ3.*t4.*t7.*t8.*t10-dQ1.*dQ2.*m6.*t2.*t5.*t8.*t17.*2.0-dQ1.*dQ2.*m6.*t3.*t5.*t7.*t17.*2.0-dQ1.*dQ3.*m6.*t2.*t5.*t8.*t17.*2.0-dQ1.*dQ3.*m6.*t3.*t5.*t7.*t17.*2.0;
et545 = dQ2.*dQ3.*m6.*t4.*t5.*t9.*t17.*-2.0-dQ1.*dQ5.*m6.*t2.*t3.*t10.*t20.*2.0+dQ2.*dQ3.*m6.*t4.*t5.*t9.*t20.*2.0+dQ2.*dQ5.*m6.*t4.*t6.*t11.*t17.*2.0+dQ3.*dQ5.*m6.*t4.*t6.*t11.*t17.*2.0-dQ2.*dQ5.*m6.*t4.*t6.*t11.*t20.*2.0-dQ3.*dQ5.*m6.*t4.*t6.*t11.*t20.*2.0+dQ1.*dQ5.*m6.*t7.*t8.*t10.*t20.*2.0+dQ2.*dQ3.*m6.*t6.*t11.*t17.*t34.*2.0-dQ2.*dQ4.*m6.*t4.*t10.*t17.*t36.*2.0-dQ2.*dQ3.*m6.*t6.*t11.*t17.*t35.*2.0+dQ2.*dQ5.*m6.*t5.*t9.*t17.*t36.*2.0-dQ3.*dQ4.*m6.*t4.*t10.*t17.*t36.*2.0+dQ3.*dQ5.*m6.*t5.*t9.*t17.*t36.*2.0-dQ2.*dQ3.*m6.*t6.*t11.*t20.*t34.*2.0+dQ2.*dQ4.*m6.*t4.*t10.*t20.*t36.*2.0+dQ2.*dQ3.*m6.*t6.*t11.*t20.*t35.*2.0-dQ2.*dQ5.*m6.*t5.*t9.*t20.*t36.*2.0+dQ3.*dQ4.*m6.*t4.*t10.*t20.*t36.*2.0-dQ3.*dQ5.*m6.*t5.*t9.*t20.*t36.*2.0;
et546 = Lx2.*Lxcm6.*dQ1.*dQ2.*m6.*t4.*t6.*t7.*-2.0+Lx3.*Lxcm6.*dQ2.*dQ3.*m6.*t4.*t5.*t11.*2.0+Lx3.*Lycm6.*dQ2.*dQ3.*m6.*t4.*t5.*t6.*2.0+Lx2.*Lycm6.*dQ1.*dQ2.*m6.*t4.*t7.*t11.*2.0-Lxcm6.*Lycm6.*dQ1.*dQ5.*m6.*t2.*t8.*t9.*2.0-Lxcm6.*Lycm6.*dQ1.*dQ5.*m6.*t3.*t7.*t9.*2.0-Lxcm6.*Lycm6.*dQ2.*dQ4.*m6.*t5.*t9.*t10.*2.0-Lxcm6.*Lycm6.*dQ3.*dQ4.*m6.*t5.*t9.*t10.*2.0+Lxcm6.*Lycm6.*dQ4.*dQ5.*m6.*t6.*t10.*t11.*4.0-Lxcm6.*Lycm6.*dQ1.*dQ4.*m6.*t2.*t3.*t35.*2.0-Lxcm6.*Lycm6.*dQ1.*dQ4.*m6.*t2.*t3.*t36.*4.0+Lxcm6.*Lycm6.*dQ1.*dQ4.*m6.*t7.*t8.*t35.*2.0+Lxcm6.*Lycm6.*dQ1.*dQ4.*m6.*t7.*t8.*t36.*4.0+Lxcm6.*Lycm6.*dQ2.*dQ3.*m6.*t34.*t35.*t36.*4.0-Lxcm6.*Lz5.*dQ2.*dQ3.*m6.*t5.*t10.*t11.*2.0-Lxcm6.*Lz5.*dQ2.*dQ4.*m6.*t9.*t11.*t35.*2.0-Lxcm6.*Lz5.*dQ3.*dQ4.*m6.*t9.*t11.*t35.*2.0-Lxcm6.*Lzcm6.*dQ2.*dQ3.*m6.*t5.*t10.*t11.*2.0;
et547 = Lxcm6.*Lzcm6.*dQ2.*dQ4.*m6.*t9.*t11.*t35.*-2.0-Lxcm6.*Lzcm6.*dQ3.*dQ4.*m6.*t9.*t11.*t35.*2.0-Lycm6.*Lz5.*dQ2.*dQ3.*m6.*t5.*t6.*t10.*2.0-Lycm6.*Lz5.*dQ2.*dQ5.*m6.*t9.*t10.*t11.*2.0-Lycm6.*Lz5.*dQ3.*dQ5.*m6.*t9.*t10.*t11.*2.0-Lycm6.*Lz5.*dQ2.*dQ4.*m6.*t6.*t9.*t35.*2.0-Lycm6.*Lz5.*dQ3.*dQ4.*m6.*t6.*t9.*t35.*2.0-Lycm6.*Lzcm6.*dQ2.*dQ3.*m6.*t5.*t6.*t10.*2.0-Lycm6.*Lzcm6.*dQ2.*dQ5.*m6.*t9.*t10.*t11.*2.0-Lycm6.*Lzcm6.*dQ3.*dQ5.*m6.*t9.*t10.*t11.*2.0-Lycm6.*Lzcm6.*dQ2.*dQ4.*m6.*t6.*t9.*t35.*2.0-Lycm6.*Lzcm6.*dQ3.*dQ4.*m6.*t6.*t9.*t35.*2.0-Ixx6.*dQ1.*dQ5.*t2.*t6.*t8.*t9.*t11.*2.0-Ixx6.*dQ1.*dQ5.*t3.*t6.*t7.*t9.*t11.*2.0-Ixx6.*dQ2.*dQ4.*t5.*t6.*t9.*t10.*t11.*2.0-Ixx6.*dQ3.*dQ4.*t5.*t6.*t9.*t10.*t11.*2.0+Ixx6.*dQ1.*dQ2.*t2.*t3.*t4.*t10.*t36.*2.0+Ixx6.*dQ1.*dQ3.*t2.*t3.*t4.*t10.*t36.*2.0;
et548 = Ixx6.*dQ1.*dQ5.*t2.*t4.*t5.*t8.*t36.*2.0+Ixx6.*dQ1.*dQ5.*t3.*t4.*t5.*t7.*t36.*2.0-Ixx6.*dQ1.*dQ4.*t2.*t3.*t6.*t11.*t35.*2.0-Ixx6.*dQ1.*dQ2.*t4.*t7.*t8.*t10.*t36.*2.0-Ixx6.*dQ1.*dQ3.*t4.*t7.*t8.*t10.*t36.*2.0+Ixx6.*dQ1.*dQ4.*t6.*t7.*t8.*t11.*t35.*2.0+Ixx6.*dQ1.*dQ2.*t2.*t5.*t8.*t34.*t36.*4.0+Ixx6.*dQ1.*dQ2.*t3.*t5.*t7.*t34.*t36.*4.0+Ixx6.*dQ1.*dQ3.*t2.*t5.*t8.*t34.*t36.*4.0+Ixx6.*dQ1.*dQ3.*t3.*t5.*t7.*t34.*t36.*4.0-Ixy6.*dQ1.*dQ2.*t2.*t3.*t5.*t9.*t10-Ixy6.*dQ1.*dQ3.*t2.*t3.*t5.*t9.*t10+Ixy6.*dQ1.*dQ4.*t2.*t4.*t5.*t8.*t10+Ixy6.*dQ1.*dQ4.*t3.*t4.*t5.*t7.*t10-Ixy6.*dQ1.*dQ2.*t2.*t5.*t6.*t8.*t11.*2.0-Ixy6.*dQ1.*dQ2.*t3.*t5.*t6.*t7.*t11.*2.0-Ixy6.*dQ1.*dQ3.*t2.*t5.*t6.*t8.*t11.*2.0-Ixy6.*dQ1.*dQ3.*t3.*t5.*t6.*t7.*t11.*2.0+Ixy6.*dQ1.*dQ5.*t2.*t3.*t6.*t10.*t11.*2.0;
et549 = Ixy6.*dQ2.*dQ3.*t4.*t5.*t6.*t9.*t11.*-4.0+Ixy6.*dQ1.*dQ2.*t5.*t7.*t8.*t9.*t10+Ixy6.*dQ1.*dQ3.*t5.*t7.*t8.*t9.*t10-Ixy6.*dQ1.*dQ5.*t6.*t7.*t8.*t10.*t11.*2.0-Ixy6.*dQ1.*dQ2.*t2.*t4.*t8.*t9.*t35-Ixy6.*dQ1.*dQ2.*t3.*t4.*t7.*t9.*t35+Ixy6.*dQ1.*dQ2.*t2.*t4.*t8.*t9.*t36.*2.0+Ixy6.*dQ1.*dQ2.*t3.*t4.*t7.*t9.*t36.*2.0-Ixy6.*dQ1.*dQ3.*t2.*t4.*t8.*t9.*t35-Ixy6.*dQ1.*dQ3.*t3.*t4.*t7.*t9.*t35+Ixy6.*dQ1.*dQ3.*t2.*t4.*t8.*t9.*t36.*2.0+Ixy6.*dQ1.*dQ3.*t3.*t4.*t7.*t9.*t36.*2.0+Ixz6.*dQ1.*dQ2.*t2.*t3.*t4.*t5.*t6+Ixz6.*dQ1.*dQ3.*t2.*t3.*t4.*t5.*t6-Ixz6.*dQ1.*dQ2.*t4.*t5.*t6.*t7.*t8-Ixz6.*dQ1.*dQ3.*t4.*t5.*t6.*t7.*t8+Ixz6.*dQ1.*dQ4.*t2.*t3.*t5.*t10.*t11-Ixz6.*dQ1.*dQ5.*t2.*t4.*t6.*t8.*t10-Ixz6.*dQ1.*dQ5.*t3.*t4.*t6.*t7.*t10;
et550 = -Ixz6.*dQ1.*dQ4.*t5.*t7.*t8.*t10.*t11-Ixz6.*dQ1.*dQ2.*t2.*t3.*t9.*t11.*t35-Ixz6.*dQ1.*dQ2.*t2.*t6.*t8.*t10.*t34-Ixz6.*dQ1.*dQ2.*t3.*t6.*t7.*t10.*t34-Ixz6.*dQ1.*dQ3.*t2.*t3.*t9.*t11.*t35-Ixz6.*dQ1.*dQ3.*t2.*t6.*t8.*t10.*t34-Ixz6.*dQ1.*dQ3.*t3.*t6.*t7.*t10.*t34+Ixz6.*dQ1.*dQ4.*t2.*t4.*t8.*t11.*t35+Ixz6.*dQ1.*dQ4.*t3.*t4.*t7.*t11.*t35+Ixz6.*dQ1.*dQ2.*t7.*t8.*t9.*t11.*t35+Ixz6.*dQ1.*dQ3.*t7.*t8.*t9.*t11.*t35-Iyx6.*dQ1.*dQ2.*t2.*t3.*t5.*t9.*t10-Iyx6.*dQ1.*dQ3.*t2.*t3.*t5.*t9.*t10+Iyx6.*dQ1.*dQ4.*t2.*t4.*t5.*t8.*t10+Iyx6.*dQ1.*dQ4.*t3.*t4.*t5.*t7.*t10-Iyx6.*dQ1.*dQ2.*t2.*t5.*t6.*t8.*t11.*2.0-Iyx6.*dQ1.*dQ2.*t3.*t5.*t6.*t7.*t11.*2.0-Iyx6.*dQ1.*dQ3.*t2.*t5.*t6.*t8.*t11.*2.0-Iyx6.*dQ1.*dQ3.*t3.*t5.*t6.*t7.*t11.*2.0;
et551 = Iyx6.*dQ1.*dQ5.*t2.*t3.*t6.*t10.*t11.*2.0-Iyx6.*dQ2.*dQ3.*t4.*t5.*t6.*t9.*t11.*4.0+Iyx6.*dQ1.*dQ2.*t5.*t7.*t8.*t9.*t10+Iyx6.*dQ1.*dQ3.*t5.*t7.*t8.*t9.*t10-Iyx6.*dQ1.*dQ5.*t6.*t7.*t8.*t10.*t11.*2.0-Iyx6.*dQ1.*dQ2.*t2.*t4.*t8.*t9.*t35-Iyx6.*dQ1.*dQ2.*t3.*t4.*t7.*t9.*t35+Iyx6.*dQ1.*dQ2.*t2.*t4.*t8.*t9.*t36.*2.0+Iyx6.*dQ1.*dQ2.*t3.*t4.*t7.*t9.*t36.*2.0-Iyx6.*dQ1.*dQ3.*t2.*t4.*t8.*t9.*t35-Iyx6.*dQ1.*dQ3.*t3.*t4.*t7.*t9.*t35+Iyx6.*dQ1.*dQ3.*t2.*t4.*t8.*t9.*t36.*2.0+Iyx6.*dQ1.*dQ3.*t3.*t4.*t7.*t9.*t36.*2.0+Iyy6.*dQ1.*dQ5.*t2.*t6.*t8.*t9.*t11.*2.0+Iyy6.*dQ1.*dQ5.*t3.*t6.*t7.*t9.*t11.*2.0-Iyy6.*dQ1.*dQ2.*t2.*t3.*t4.*t10.*t36.*2.0-Iyy6.*dQ1.*dQ3.*t2.*t3.*t4.*t10.*t36.*2.0-Iyy6.*dQ1.*dQ5.*t2.*t4.*t5.*t8.*t36.*2.0-Iyy6.*dQ1.*dQ5.*t3.*t4.*t5.*t7.*t36.*2.0;
et552 = Iyy6.*dQ1.*dQ4.*t2.*t3.*t6.*t11.*t35.*2.0+Iyy6.*dQ1.*dQ2.*t4.*t7.*t8.*t10.*t36.*2.0+Iyy6.*dQ1.*dQ3.*t4.*t7.*t8.*t10.*t36.*2.0-Iyy6.*dQ1.*dQ4.*t6.*t7.*t8.*t11.*t35.*2.0-Iyy6.*dQ1.*dQ2.*t2.*t5.*t8.*t34.*t36.*4.0-Iyy6.*dQ1.*dQ2.*t3.*t5.*t7.*t34.*t36.*4.0-Iyy6.*dQ1.*dQ3.*t2.*t5.*t8.*t34.*t36.*4.0-Iyy6.*dQ1.*dQ3.*t3.*t5.*t7.*t34.*t36.*4.0-Iyz6.*dQ1.*dQ2.*t2.*t3.*t4.*t5.*t11-Iyz6.*dQ1.*dQ3.*t2.*t3.*t4.*t5.*t11+Iyz6.*dQ1.*dQ4.*t2.*t3.*t5.*t6.*t10+Iyz6.*dQ1.*dQ2.*t4.*t5.*t7.*t8.*t11+Iyz6.*dQ1.*dQ3.*t4.*t5.*t7.*t8.*t11-Iyz6.*dQ1.*dQ4.*t5.*t6.*t7.*t8.*t10+Iyz6.*dQ1.*dQ5.*t2.*t4.*t8.*t10.*t11+Iyz6.*dQ1.*dQ5.*t3.*t4.*t7.*t10.*t11-Iyz6.*dQ1.*dQ2.*t2.*t3.*t6.*t9.*t35-Iyz6.*dQ1.*dQ3.*t2.*t3.*t6.*t9.*t35+Iyz6.*dQ1.*dQ4.*t2.*t4.*t6.*t8.*t35;
et553 = Iyz6.*dQ1.*dQ4.*t3.*t4.*t6.*t7.*t35+Iyz6.*dQ1.*dQ2.*t2.*t8.*t10.*t11.*t34+Iyz6.*dQ1.*dQ2.*t3.*t7.*t10.*t11.*t34+Iyz6.*dQ1.*dQ2.*t6.*t7.*t8.*t9.*t35+Iyz6.*dQ1.*dQ3.*t2.*t8.*t10.*t11.*t34+Iyz6.*dQ1.*dQ3.*t3.*t7.*t10.*t11.*t34+Iyz6.*dQ1.*dQ3.*t6.*t7.*t8.*t9.*t35+Izx6.*dQ1.*dQ2.*t2.*t3.*t4.*t5.*t6+Izx6.*dQ1.*dQ3.*t2.*t3.*t4.*t5.*t6-Izx6.*dQ1.*dQ2.*t4.*t5.*t6.*t7.*t8-Izx6.*dQ1.*dQ3.*t4.*t5.*t6.*t7.*t8+Izx6.*dQ1.*dQ4.*t2.*t3.*t5.*t10.*t11-Izx6.*dQ1.*dQ5.*t2.*t4.*t6.*t8.*t10-Izx6.*dQ1.*dQ5.*t3.*t4.*t6.*t7.*t10-Izx6.*dQ1.*dQ4.*t5.*t7.*t8.*t10.*t11-Izx6.*dQ1.*dQ2.*t2.*t3.*t9.*t11.*t35-Izx6.*dQ1.*dQ2.*t2.*t6.*t8.*t10.*t34-Izx6.*dQ1.*dQ2.*t3.*t6.*t7.*t10.*t34-Izx6.*dQ1.*dQ3.*t2.*t3.*t9.*t11.*t35-Izx6.*dQ1.*dQ3.*t2.*t6.*t8.*t10.*t34;
et554 = -Izx6.*dQ1.*dQ3.*t3.*t6.*t7.*t10.*t34+Izx6.*dQ1.*dQ4.*t2.*t4.*t8.*t11.*t35+Izx6.*dQ1.*dQ4.*t3.*t4.*t7.*t11.*t35+Izx6.*dQ1.*dQ2.*t7.*t8.*t9.*t11.*t35+Izx6.*dQ1.*dQ3.*t7.*t8.*t9.*t11.*t35-Izy6.*dQ1.*dQ2.*t2.*t3.*t4.*t5.*t11-Izy6.*dQ1.*dQ3.*t2.*t3.*t4.*t5.*t11+Izy6.*dQ1.*dQ4.*t2.*t3.*t5.*t6.*t10+Izy6.*dQ1.*dQ2.*t4.*t5.*t7.*t8.*t11+Izy6.*dQ1.*dQ3.*t4.*t5.*t7.*t8.*t11-Izy6.*dQ1.*dQ4.*t5.*t6.*t7.*t8.*t10+Izy6.*dQ1.*dQ5.*t2.*t4.*t8.*t10.*t11+Izy6.*dQ1.*dQ5.*t3.*t4.*t7.*t10.*t11-Izy6.*dQ1.*dQ2.*t2.*t3.*t6.*t9.*t35-Izy6.*dQ1.*dQ3.*t2.*t3.*t6.*t9.*t35+Izy6.*dQ1.*dQ4.*t2.*t4.*t6.*t8.*t35+Izy6.*dQ1.*dQ4.*t3.*t4.*t6.*t7.*t35+Izy6.*dQ1.*dQ2.*t2.*t8.*t10.*t11.*t34+Izy6.*dQ1.*dQ2.*t3.*t7.*t10.*t11.*t34+Izy6.*dQ1.*dQ2.*t6.*t7.*t8.*t9.*t35;
et555 = Izy6.*dQ1.*dQ3.*t2.*t8.*t10.*t11.*t34+Izy6.*dQ1.*dQ3.*t3.*t7.*t10.*t11.*t34+Izy6.*dQ1.*dQ3.*t6.*t7.*t8.*t9.*t35-dQ1.*dQ2.*m6.*t2.*t3.*t4.*t10.*t20.*2.0-dQ1.*dQ3.*m6.*t2.*t3.*t4.*t10.*t20.*2.0-dQ1.*dQ4.*m6.*t2.*t3.*t6.*t11.*t17.*2.0-dQ1.*dQ5.*m6.*t2.*t4.*t5.*t8.*t20.*2.0-dQ1.*dQ5.*m6.*t3.*t4.*t5.*t7.*t20.*2.0+dQ1.*dQ4.*m6.*t2.*t3.*t6.*t11.*t20.*2.0+dQ1.*dQ2.*m6.*t4.*t7.*t8.*t10.*t20.*2.0+dQ1.*dQ3.*m6.*t4.*t7.*t8.*t10.*t20.*2.0+dQ1.*dQ4.*m6.*t6.*t7.*t8.*t11.*t17.*2.0-dQ1.*dQ4.*m6.*t6.*t7.*t8.*t11.*t20.*2.0+dQ1.*dQ2.*m6.*t2.*t5.*t8.*t17.*t34.*2.0+dQ1.*dQ2.*m6.*t3.*t5.*t7.*t17.*t34.*2.0+dQ1.*dQ3.*m6.*t2.*t5.*t8.*t17.*t34.*2.0+dQ1.*dQ3.*m6.*t3.*t5.*t7.*t17.*t34.*2.0+dQ1.*dQ2.*m6.*t2.*t5.*t8.*t17.*t36.*2.0+dQ1.*dQ2.*m6.*t3.*t5.*t7.*t17.*t36.*2.0;
et556 = dQ1.*dQ2.*m6.*t2.*t5.*t8.*t20.*t34.*-2.0-dQ1.*dQ2.*m6.*t3.*t5.*t7.*t20.*t34.*2.0+dQ1.*dQ3.*m6.*t2.*t5.*t8.*t17.*t36.*2.0+dQ1.*dQ3.*m6.*t3.*t5.*t7.*t17.*t36.*2.0-dQ1.*dQ3.*m6.*t2.*t5.*t8.*t20.*t34.*2.0-dQ1.*dQ3.*m6.*t3.*t5.*t7.*t20.*t34.*2.0-dQ1.*dQ2.*m6.*t2.*t5.*t8.*t20.*t36.*2.0-dQ1.*dQ2.*m6.*t3.*t5.*t7.*t20.*t36.*2.0-dQ1.*dQ5.*m6.*t2.*t3.*t10.*t17.*t36.*2.0-dQ1.*dQ3.*m6.*t2.*t5.*t8.*t20.*t36.*2.0-dQ1.*dQ3.*m6.*t3.*t5.*t7.*t20.*t36.*2.0+dQ2.*dQ3.*m6.*t4.*t5.*t9.*t17.*t36.*4.0+dQ1.*dQ5.*m6.*t2.*t3.*t10.*t20.*t36.*2.0-dQ2.*dQ3.*m6.*t4.*t5.*t9.*t20.*t36.*4.0+dQ1.*dQ5.*m6.*t7.*t8.*t10.*t17.*t36.*2.0-dQ1.*dQ5.*m6.*t7.*t8.*t10.*t20.*t36.*2.0+dQ2.*dQ3.*m6.*t6.*t11.*t17.*t34.*t35.*2.0-dQ2.*dQ3.*m6.*t6.*t11.*t20.*t34.*t35.*2.0;
et557 = Ixx6.*dQ1.*dQ2.*t2.*t4.*t6.*t8.*t9.*t11.*-2.0-Ixx6.*dQ1.*dQ2.*t3.*t4.*t6.*t7.*t9.*t11.*2.0-Ixx6.*dQ1.*dQ3.*t2.*t4.*t6.*t8.*t9.*t11.*2.0-Ixx6.*dQ1.*dQ3.*t3.*t4.*t6.*t7.*t9.*t11.*2.0+Ixy6.*dQ1.*dQ2.*t2.*t3.*t4.*t6.*t10.*t11.*2.0+Ixy6.*dQ1.*dQ3.*t2.*t3.*t4.*t6.*t10.*t11.*2.0+Ixy6.*dQ1.*dQ5.*t2.*t4.*t5.*t6.*t8.*t11.*2.0+Ixy6.*dQ1.*dQ5.*t3.*t4.*t5.*t6.*t7.*t11.*2.0-Ixy6.*dQ1.*dQ2.*t4.*t6.*t7.*t8.*t10.*t11.*2.0-Ixy6.*dQ1.*dQ3.*t4.*t6.*t7.*t8.*t10.*t11.*2.0+Ixy6.*dQ1.*dQ2.*t2.*t3.*t5.*t9.*t10.*t36.*2.0+Ixy6.*dQ1.*dQ2.*t2.*t5.*t6.*t8.*t11.*t34.*4.0+Ixy6.*dQ1.*dQ2.*t3.*t5.*t6.*t7.*t11.*t34.*4.0+Ixy6.*dQ1.*dQ3.*t2.*t3.*t5.*t9.*t10.*t36.*2.0+Ixy6.*dQ1.*dQ3.*t2.*t5.*t6.*t8.*t11.*t34.*4.0+Ixy6.*dQ1.*dQ3.*t3.*t5.*t6.*t7.*t11.*t34.*4.0-Ixy6.*dQ1.*dQ4.*t2.*t4.*t5.*t8.*t10.*t36.*2.0;
et558 = Ixy6.*dQ1.*dQ4.*t3.*t4.*t5.*t7.*t10.*t36.*-2.0-Ixy6.*dQ1.*dQ2.*t5.*t7.*t8.*t9.*t10.*t36.*2.0-Ixy6.*dQ1.*dQ3.*t5.*t7.*t8.*t9.*t10.*t36.*2.0+Ixy6.*dQ1.*dQ2.*t2.*t4.*t8.*t9.*t35.*t36.*2.0+Ixy6.*dQ1.*dQ2.*t3.*t4.*t7.*t9.*t35.*t36.*2.0+Ixy6.*dQ1.*dQ3.*t2.*t4.*t8.*t9.*t35.*t36.*2.0+Ixy6.*dQ1.*dQ3.*t3.*t4.*t7.*t9.*t35.*t36.*2.0+Iyx6.*dQ1.*dQ2.*t2.*t3.*t4.*t6.*t10.*t11.*2.0+Iyx6.*dQ1.*dQ3.*t2.*t3.*t4.*t6.*t10.*t11.*2.0+Iyx6.*dQ1.*dQ5.*t2.*t4.*t5.*t6.*t8.*t11.*2.0+Iyx6.*dQ1.*dQ5.*t3.*t4.*t5.*t6.*t7.*t11.*2.0-Iyx6.*dQ1.*dQ2.*t4.*t6.*t7.*t8.*t10.*t11.*2.0-Iyx6.*dQ1.*dQ3.*t4.*t6.*t7.*t8.*t10.*t11.*2.0+Iyx6.*dQ1.*dQ2.*t2.*t3.*t5.*t9.*t10.*t36.*2.0+Iyx6.*dQ1.*dQ2.*t2.*t5.*t6.*t8.*t11.*t34.*4.0+Iyx6.*dQ1.*dQ2.*t3.*t5.*t6.*t7.*t11.*t34.*4.0+Iyx6.*dQ1.*dQ3.*t2.*t3.*t5.*t9.*t10.*t36.*2.0;
et559 = Iyx6.*dQ1.*dQ3.*t2.*t5.*t6.*t8.*t11.*t34.*4.0+Iyx6.*dQ1.*dQ3.*t3.*t5.*t6.*t7.*t11.*t34.*4.0-Iyx6.*dQ1.*dQ4.*t2.*t4.*t5.*t8.*t10.*t36.*2.0-Iyx6.*dQ1.*dQ4.*t3.*t4.*t5.*t7.*t10.*t36.*2.0-Iyx6.*dQ1.*dQ2.*t5.*t7.*t8.*t9.*t10.*t36.*2.0-Iyx6.*dQ1.*dQ3.*t5.*t7.*t8.*t9.*t10.*t36.*2.0+Iyx6.*dQ1.*dQ2.*t2.*t4.*t8.*t9.*t35.*t36.*2.0+Iyx6.*dQ1.*dQ2.*t3.*t4.*t7.*t9.*t35.*t36.*2.0+Iyx6.*dQ1.*dQ3.*t2.*t4.*t8.*t9.*t35.*t36.*2.0+Iyx6.*dQ1.*dQ3.*t3.*t4.*t7.*t9.*t35.*t36.*2.0+Iyy6.*dQ1.*dQ2.*t2.*t4.*t6.*t8.*t9.*t11.*2.0+Iyy6.*dQ1.*dQ2.*t3.*t4.*t6.*t7.*t9.*t11.*2.0+Iyy6.*dQ1.*dQ3.*t2.*t4.*t6.*t8.*t9.*t11.*2.0+Iyy6.*dQ1.*dQ3.*t3.*t4.*t6.*t7.*t9.*t11.*2.0+dQ1.*dQ5.*m6.*t2.*t6.*t8.*t9.*t11.*t17.*2.0+dQ1.*dQ5.*m6.*t3.*t6.*t7.*t9.*t11.*t17.*2.0-dQ1.*dQ5.*m6.*t2.*t6.*t8.*t9.*t11.*t20.*2.0;
et560 = dQ1.*dQ5.*m6.*t3.*t6.*t7.*t9.*t11.*t20.*-2.0-dQ2.*dQ4.*m6.*t5.*t6.*t9.*t10.*t11.*t20.*2.0-dQ3.*dQ4.*m6.*t5.*t6.*t9.*t10.*t11.*t20.*2.0-dQ1.*dQ2.*m6.*t2.*t3.*t4.*t10.*t17.*t36.*2.0-dQ1.*dQ3.*m6.*t2.*t3.*t4.*t10.*t17.*t36.*2.0+dQ1.*dQ2.*m6.*t2.*t3.*t4.*t10.*t20.*t36.*2.0-dQ1.*dQ5.*m6.*t2.*t4.*t5.*t8.*t17.*t36.*2.0-dQ1.*dQ5.*m6.*t3.*t4.*t5.*t7.*t17.*t36.*2.0+dQ1.*dQ3.*m6.*t2.*t3.*t4.*t10.*t20.*t36.*2.0+dQ1.*dQ4.*m6.*t2.*t3.*t6.*t11.*t17.*t35.*2.0+dQ1.*dQ5.*m6.*t2.*t4.*t5.*t8.*t20.*t36.*2.0+dQ1.*dQ5.*m6.*t3.*t4.*t5.*t7.*t20.*t36.*2.0-dQ1.*dQ4.*m6.*t2.*t3.*t6.*t11.*t20.*t35.*2.0+dQ1.*dQ2.*m6.*t4.*t7.*t8.*t10.*t17.*t36.*2.0+dQ1.*dQ3.*m6.*t4.*t7.*t8.*t10.*t17.*t36.*2.0-dQ1.*dQ2.*m6.*t4.*t7.*t8.*t10.*t20.*t36.*2.0-dQ1.*dQ3.*m6.*t4.*t7.*t8.*t10.*t20.*t36.*2.0;
et561 = dQ1.*dQ4.*m6.*t6.*t7.*t8.*t11.*t17.*t35.*-2.0+dQ1.*dQ4.*m6.*t6.*t7.*t8.*t11.*t20.*t35.*2.0-dQ1.*dQ2.*m6.*t2.*t5.*t8.*t17.*t34.*t36.*4.0-dQ1.*dQ2.*m6.*t3.*t5.*t7.*t17.*t34.*t36.*4.0-dQ1.*dQ3.*m6.*t2.*t5.*t8.*t17.*t34.*t36.*4.0-dQ1.*dQ3.*m6.*t3.*t5.*t7.*t17.*t34.*t36.*4.0+dQ1.*dQ2.*m6.*t2.*t5.*t8.*t20.*t34.*t36.*4.0+dQ1.*dQ2.*m6.*t3.*t5.*t7.*t20.*t34.*t36.*4.0+dQ1.*dQ3.*m6.*t2.*t5.*t8.*t20.*t34.*t36.*4.0+dQ1.*dQ3.*m6.*t3.*t5.*t7.*t20.*t34.*t36.*4.0-Lx3.*Lxcm6.*dQ1.*dQ2.*m6.*t2.*t4.*t6.*t8.*2.0-Lx3.*Lxcm6.*dQ1.*dQ2.*m6.*t3.*t4.*t6.*t7.*2.0-Lx3.*Lxcm6.*dQ1.*dQ3.*m6.*t2.*t4.*t6.*t8.*2.0-Lx3.*Lxcm6.*dQ1.*dQ3.*m6.*t3.*t4.*t6.*t7.*2.0+Lx2.*Lxcm6.*dQ1.*dQ2.*m6.*t5.*t7.*t9.*t11.*2.0+Lx3.*Lycm6.*dQ1.*dQ2.*m6.*t2.*t4.*t8.*t11.*2.0+Lx3.*Lycm6.*dQ1.*dQ2.*m6.*t3.*t4.*t7.*t11.*2.0;
et562 = Lx2.*Lycm6.*dQ1.*dQ2.*m6.*t5.*t6.*t7.*t9.*2.0+Lx3.*Lycm6.*dQ1.*dQ3.*m6.*t2.*t4.*t8.*t11.*2.0+Lx3.*Lycm6.*dQ1.*dQ3.*m6.*t3.*t4.*t7.*t11.*2.0-Lxcm6.*Lycm6.*dQ1.*dQ2.*m6.*t2.*t4.*t8.*t9.*2.0-Lxcm6.*Lycm6.*dQ1.*dQ2.*m6.*t3.*t4.*t7.*t9.*2.0-Lxcm6.*Lycm6.*dQ1.*dQ3.*m6.*t2.*t4.*t8.*t9.*2.0-Lxcm6.*Lycm6.*dQ1.*dQ3.*m6.*t3.*t4.*t7.*t9.*2.0+Lxcm6.*Lycm6.*dQ2.*dQ4.*m6.*t4.*t6.*t10.*t11.*4.0-Lxcm6.*Lycm6.*dQ2.*dQ5.*m6.*t5.*t6.*t9.*t11.*4.0+Lxcm6.*Lycm6.*dQ3.*dQ4.*m6.*t4.*t6.*t10.*t11.*4.0-Lxcm6.*Lycm6.*dQ3.*dQ5.*m6.*t5.*t6.*t9.*t11.*4.0+Lxcm6.*Lycm6.*dQ1.*dQ5.*m6.*t2.*t8.*t9.*t36.*4.0+Lxcm6.*Lycm6.*dQ1.*dQ5.*m6.*t3.*t7.*t9.*t36.*4.0+Lxcm6.*Lycm6.*dQ1.*dQ4.*m6.*t2.*t3.*t35.*t36.*4.0-Lxcm6.*Lycm6.*dQ1.*dQ4.*m6.*t7.*t8.*t35.*t36.*4.0+Lxcm6.*Lz4.*dQ1.*dQ2.*m6.*t2.*t3.*t4.*t6.*2.0+Lxcm6.*Lz4.*dQ1.*dQ3.*m6.*t2.*t3.*t4.*t6.*2.0;
et563 = Lxcm6.*Lz5.*dQ1.*dQ5.*m6.*t2.*t3.*t5.*t6.*2.0-Lxcm6.*Lz4.*dQ1.*dQ2.*m6.*t4.*t6.*t7.*t8.*2.0-Lxcm6.*Lz4.*dQ1.*dQ3.*m6.*t4.*t6.*t7.*t8.*2.0-Lxcm6.*Lz5.*dQ1.*dQ4.*m6.*t2.*t4.*t8.*t11.*2.0-Lxcm6.*Lz5.*dQ1.*dQ4.*m6.*t3.*t4.*t7.*t11.*2.0-Lxcm6.*Lz5.*dQ1.*dQ5.*m6.*t5.*t6.*t7.*t8.*2.0+Lxcm6.*Lz5.*dQ2.*dQ3.*m6.*t4.*t6.*t9.*t10.*2.0+Lxcm6.*Lz5.*dQ2.*dQ3.*m6.*t5.*t10.*t11.*t34.*2.0+Lxcm6.*Lzcm6.*dQ1.*dQ5.*m6.*t2.*t3.*t5.*t6.*2.0-Lxcm6.*Lzcm6.*dQ1.*dQ4.*m6.*t2.*t4.*t8.*t11.*2.0-Lxcm6.*Lzcm6.*dQ1.*dQ4.*m6.*t3.*t4.*t7.*t11.*2.0-Lxcm6.*Lzcm6.*dQ1.*dQ5.*m6.*t5.*t6.*t7.*t8.*2.0+Lxcm6.*Lzcm6.*dQ2.*dQ3.*m6.*t4.*t6.*t9.*t10.*2.0+Lxcm6.*Lzcm6.*dQ2.*dQ3.*m6.*t5.*t10.*t11.*t34.*2.0-Lycm6.*Lz4.*dQ1.*dQ2.*m6.*t2.*t3.*t4.*t11.*2.0-Lycm6.*Lz4.*dQ1.*dQ3.*m6.*t2.*t3.*t4.*t11.*2.0-Lycm6.*Lz5.*dQ1.*dQ4.*m6.*t2.*t4.*t6.*t8.*2.0;
et564 = Lycm6.*Lz5.*dQ1.*dQ4.*m6.*t3.*t4.*t6.*t7.*-2.0-Lycm6.*Lz5.*dQ1.*dQ5.*m6.*t2.*t3.*t5.*t11.*2.0+Lycm6.*Lz4.*dQ1.*dQ2.*m6.*t4.*t7.*t8.*t11.*2.0+Lycm6.*Lz4.*dQ1.*dQ3.*m6.*t4.*t7.*t8.*t11.*2.0+Lycm6.*Lz5.*dQ1.*dQ5.*m6.*t5.*t7.*t8.*t11.*2.0-Lycm6.*Lz5.*dQ2.*dQ3.*m6.*t4.*t9.*t10.*t11.*2.0+Lycm6.*Lz5.*dQ2.*dQ3.*m6.*t5.*t6.*t10.*t34.*2.0-Lycm6.*Lzcm6.*dQ1.*dQ4.*m6.*t2.*t4.*t6.*t8.*2.0-Lycm6.*Lzcm6.*dQ1.*dQ4.*m6.*t3.*t4.*t6.*t7.*2.0-Lycm6.*Lzcm6.*dQ1.*dQ5.*m6.*t2.*t3.*t5.*t11.*2.0+Lycm6.*Lzcm6.*dQ1.*dQ5.*m6.*t5.*t7.*t8.*t11.*2.0-Lycm6.*Lzcm6.*dQ2.*dQ3.*m6.*t4.*t9.*t10.*t11.*2.0+Lycm6.*Lzcm6.*dQ2.*dQ3.*m6.*t5.*t6.*t10.*t34.*2.0+Lx3.*Lxcm6.*dQ1.*dQ2.*m6.*t2.*t5.*t8.*t9.*t11.*2.0+Lx3.*Lxcm6.*dQ1.*dQ2.*m6.*t3.*t5.*t7.*t9.*t11.*2.0+Lx3.*Lxcm6.*dQ1.*dQ3.*m6.*t2.*t5.*t8.*t9.*t11.*2.0+Lx3.*Lxcm6.*dQ1.*dQ3.*m6.*t3.*t5.*t7.*t9.*t11.*2.0;
et565 = Lx3.*Lycm6.*dQ1.*dQ2.*m6.*t2.*t5.*t6.*t8.*t9.*2.0+Lx3.*Lycm6.*dQ1.*dQ2.*m6.*t3.*t5.*t6.*t7.*t9.*2.0+Lx3.*Lycm6.*dQ1.*dQ3.*m6.*t2.*t5.*t6.*t8.*t9.*2.0+Lx3.*Lycm6.*dQ1.*dQ3.*m6.*t3.*t5.*t6.*t7.*t9.*2.0-Lxcm6.*Lycm6.*dQ1.*dQ2.*m6.*t2.*t3.*t5.*t9.*t10.*2.0-Lxcm6.*Lycm6.*dQ1.*dQ3.*m6.*t2.*t3.*t5.*t9.*t10.*2.0+Lxcm6.*Lycm6.*dQ1.*dQ4.*m6.*t2.*t4.*t5.*t8.*t10.*2.0+Lxcm6.*Lycm6.*dQ1.*dQ4.*m6.*t3.*t4.*t5.*t7.*t10.*2.0-Lxcm6.*Lycm6.*dQ1.*dQ2.*m6.*t2.*t5.*t6.*t8.*t11.*4.0-Lxcm6.*Lycm6.*dQ1.*dQ2.*m6.*t3.*t5.*t6.*t7.*t11.*4.0-Lxcm6.*Lycm6.*dQ1.*dQ3.*m6.*t2.*t5.*t6.*t8.*t11.*4.0-Lxcm6.*Lycm6.*dQ1.*dQ3.*m6.*t3.*t5.*t6.*t7.*t11.*4.0+Lxcm6.*Lycm6.*dQ1.*dQ5.*m6.*t2.*t3.*t6.*t10.*t11.*4.0-Lxcm6.*Lycm6.*dQ2.*dQ3.*m6.*t4.*t5.*t6.*t9.*t11.*8.0+Lxcm6.*Lycm6.*dQ1.*dQ2.*m6.*t5.*t7.*t8.*t9.*t10.*2.0+Lxcm6.*Lycm6.*dQ1.*dQ3.*m6.*t5.*t7.*t8.*t9.*t10.*2.0;
et566 = Lxcm6.*Lycm6.*dQ1.*dQ5.*m6.*t6.*t7.*t8.*t10.*t11.*-4.0-Lxcm6.*Lycm6.*dQ1.*dQ2.*m6.*t2.*t4.*t8.*t9.*t35.*2.0-Lxcm6.*Lycm6.*dQ1.*dQ2.*m6.*t3.*t4.*t7.*t9.*t35.*2.0+Lxcm6.*Lycm6.*dQ1.*dQ2.*m6.*t2.*t4.*t8.*t9.*t36.*4.0+Lxcm6.*Lycm6.*dQ1.*dQ2.*m6.*t3.*t4.*t7.*t9.*t36.*4.0-Lxcm6.*Lycm6.*dQ1.*dQ3.*m6.*t2.*t4.*t8.*t9.*t35.*2.0-Lxcm6.*Lycm6.*dQ1.*dQ3.*m6.*t3.*t4.*t7.*t9.*t35.*2.0+Lxcm6.*Lycm6.*dQ1.*dQ3.*m6.*t2.*t4.*t8.*t9.*t36.*4.0+Lxcm6.*Lycm6.*dQ1.*dQ3.*m6.*t3.*t4.*t7.*t9.*t36.*4.0+Lxcm6.*Lz5.*dQ1.*dQ2.*m6.*t2.*t3.*t4.*t5.*t6.*2.0+Lxcm6.*Lz5.*dQ1.*dQ3.*m6.*t2.*t3.*t4.*t5.*t6.*2.0-Lxcm6.*Lz4.*dQ1.*dQ2.*m6.*t2.*t3.*t5.*t9.*t11.*2.0-Lxcm6.*Lz4.*dQ1.*dQ3.*m6.*t2.*t3.*t5.*t9.*t11.*2.0-Lxcm6.*Lz5.*dQ1.*dQ2.*m6.*t4.*t5.*t6.*t7.*t8.*2.0-Lxcm6.*Lz5.*dQ1.*dQ3.*m6.*t4.*t5.*t6.*t7.*t8.*2.0;
et567 = Lxcm6.*Lz5.*dQ1.*dQ4.*m6.*t2.*t3.*t5.*t10.*t11.*2.0-Lxcm6.*Lz5.*dQ1.*dQ5.*m6.*t2.*t4.*t6.*t8.*t10.*2.0-Lxcm6.*Lz5.*dQ1.*dQ5.*m6.*t3.*t4.*t6.*t7.*t10.*2.0+Lxcm6.*Lz4.*dQ1.*dQ2.*m6.*t5.*t7.*t8.*t9.*t11.*2.0+Lxcm6.*Lz4.*dQ1.*dQ3.*m6.*t5.*t7.*t8.*t9.*t11.*2.0-Lxcm6.*Lz5.*dQ1.*dQ4.*m6.*t5.*t7.*t8.*t10.*t11.*2.0-Lxcm6.*Lz5.*dQ1.*dQ2.*m6.*t2.*t3.*t9.*t11.*t35.*2.0-Lxcm6.*Lz5.*dQ1.*dQ2.*m6.*t2.*t6.*t8.*t10.*t34.*2.0-Lxcm6.*Lz5.*dQ1.*dQ2.*m6.*t3.*t6.*t7.*t10.*t34.*2.0-Lxcm6.*Lz5.*dQ1.*dQ3.*m6.*t2.*t3.*t9.*t11.*t35.*2.0-Lxcm6.*Lz5.*dQ1.*dQ3.*m6.*t2.*t6.*t8.*t10.*t34.*2.0-Lxcm6.*Lz5.*dQ1.*dQ3.*m6.*t3.*t6.*t7.*t10.*t34.*2.0+Lxcm6.*Lz5.*dQ1.*dQ4.*m6.*t2.*t4.*t8.*t11.*t35.*2.0+Lxcm6.*Lz5.*dQ1.*dQ4.*m6.*t3.*t4.*t7.*t11.*t35.*2.0+Lxcm6.*Lz5.*dQ1.*dQ2.*m6.*t7.*t8.*t9.*t11.*t35.*2.0;
et568 = Lxcm6.*Lz5.*dQ1.*dQ3.*m6.*t7.*t8.*t9.*t11.*t35.*2.0+Lxcm6.*Lzcm6.*dQ1.*dQ2.*m6.*t2.*t3.*t4.*t5.*t6.*2.0+Lxcm6.*Lzcm6.*dQ1.*dQ3.*m6.*t2.*t3.*t4.*t5.*t6.*2.0-Lxcm6.*Lzcm6.*dQ1.*dQ2.*m6.*t4.*t5.*t6.*t7.*t8.*2.0-Lxcm6.*Lzcm6.*dQ1.*dQ3.*m6.*t4.*t5.*t6.*t7.*t8.*2.0+Lxcm6.*Lzcm6.*dQ1.*dQ4.*m6.*t2.*t3.*t5.*t10.*t11.*2.0-Lxcm6.*Lzcm6.*dQ1.*dQ5.*m6.*t2.*t4.*t6.*t8.*t10.*2.0-Lxcm6.*Lzcm6.*dQ1.*dQ5.*m6.*t3.*t4.*t6.*t7.*t10.*2.0-Lxcm6.*Lzcm6.*dQ1.*dQ4.*m6.*t5.*t7.*t8.*t10.*t11.*2.0-Lxcm6.*Lzcm6.*dQ1.*dQ2.*m6.*t2.*t3.*t9.*t11.*t35.*2.0-Lxcm6.*Lzcm6.*dQ1.*dQ2.*m6.*t2.*t6.*t8.*t10.*t34.*2.0-Lxcm6.*Lzcm6.*dQ1.*dQ2.*m6.*t3.*t6.*t7.*t10.*t34.*2.0-Lxcm6.*Lzcm6.*dQ1.*dQ3.*m6.*t2.*t3.*t9.*t11.*t35.*2.0-Lxcm6.*Lzcm6.*dQ1.*dQ3.*m6.*t2.*t6.*t8.*t10.*t34.*2.0-Lxcm6.*Lzcm6.*dQ1.*dQ3.*m6.*t3.*t6.*t7.*t10.*t34.*2.0;
et569 = Lxcm6.*Lzcm6.*dQ1.*dQ4.*m6.*t2.*t4.*t8.*t11.*t35.*2.0+Lxcm6.*Lzcm6.*dQ1.*dQ4.*m6.*t3.*t4.*t7.*t11.*t35.*2.0+Lxcm6.*Lzcm6.*dQ1.*dQ2.*m6.*t7.*t8.*t9.*t11.*t35.*2.0+Lxcm6.*Lzcm6.*dQ1.*dQ3.*m6.*t7.*t8.*t9.*t11.*t35.*2.0-Lycm6.*Lz4.*dQ1.*dQ2.*m6.*t2.*t3.*t5.*t6.*t9.*2.0-Lycm6.*Lz4.*dQ1.*dQ3.*m6.*t2.*t3.*t5.*t6.*t9.*2.0-Lycm6.*Lz5.*dQ1.*dQ2.*m6.*t2.*t3.*t4.*t5.*t11.*2.0-Lycm6.*Lz5.*dQ1.*dQ3.*m6.*t2.*t3.*t4.*t5.*t11.*2.0+Lycm6.*Lz5.*dQ1.*dQ4.*m6.*t2.*t3.*t5.*t6.*t10.*2.0+Lycm6.*Lz4.*dQ1.*dQ2.*m6.*t5.*t6.*t7.*t8.*t9.*2.0+Lycm6.*Lz4.*dQ1.*dQ3.*m6.*t5.*t6.*t7.*t8.*t9.*2.0+Lycm6.*Lz5.*dQ1.*dQ2.*m6.*t4.*t5.*t7.*t8.*t11.*2.0+Lycm6.*Lz5.*dQ1.*dQ3.*m6.*t4.*t5.*t7.*t8.*t11.*2.0-Lycm6.*Lz5.*dQ1.*dQ4.*m6.*t5.*t6.*t7.*t8.*t10.*2.0+Lycm6.*Lz5.*dQ1.*dQ5.*m6.*t2.*t4.*t8.*t10.*t11.*2.0+Lycm6.*Lz5.*dQ1.*dQ5.*m6.*t3.*t4.*t7.*t10.*t11.*2.0;
et570 = Lycm6.*Lz5.*dQ1.*dQ2.*m6.*t2.*t3.*t6.*t9.*t35.*-2.0-Lycm6.*Lz5.*dQ1.*dQ3.*m6.*t2.*t3.*t6.*t9.*t35.*2.0+Lycm6.*Lz5.*dQ1.*dQ4.*m6.*t2.*t4.*t6.*t8.*t35.*2.0+Lycm6.*Lz5.*dQ1.*dQ4.*m6.*t3.*t4.*t6.*t7.*t35.*2.0+Lycm6.*Lz5.*dQ1.*dQ2.*m6.*t2.*t8.*t10.*t11.*t34.*2.0+Lycm6.*Lz5.*dQ1.*dQ2.*m6.*t3.*t7.*t10.*t11.*t34.*2.0+Lycm6.*Lz5.*dQ1.*dQ2.*m6.*t6.*t7.*t8.*t9.*t35.*2.0+Lycm6.*Lz5.*dQ1.*dQ3.*m6.*t2.*t8.*t10.*t11.*t34.*2.0+Lycm6.*Lz5.*dQ1.*dQ3.*m6.*t3.*t7.*t10.*t11.*t34.*2.0+Lycm6.*Lz5.*dQ1.*dQ3.*m6.*t6.*t7.*t8.*t9.*t35.*2.0-Lycm6.*Lzcm6.*dQ1.*dQ2.*m6.*t2.*t3.*t4.*t5.*t11.*2.0-Lycm6.*Lzcm6.*dQ1.*dQ3.*m6.*t2.*t3.*t4.*t5.*t11.*2.0+Lycm6.*Lzcm6.*dQ1.*dQ4.*m6.*t2.*t3.*t5.*t6.*t10.*2.0+Lycm6.*Lzcm6.*dQ1.*dQ2.*m6.*t4.*t5.*t7.*t8.*t11.*2.0+Lycm6.*Lzcm6.*dQ1.*dQ3.*m6.*t4.*t5.*t7.*t8.*t11.*2.0-Lycm6.*Lzcm6.*dQ1.*dQ4.*m6.*t5.*t6.*t7.*t8.*t10.*2.0;
et571 = Lycm6.*Lzcm6.*dQ1.*dQ5.*m6.*t2.*t4.*t8.*t10.*t11.*2.0+Lycm6.*Lzcm6.*dQ1.*dQ5.*m6.*t3.*t4.*t7.*t10.*t11.*2.0-Lycm6.*Lzcm6.*dQ1.*dQ2.*m6.*t2.*t3.*t6.*t9.*t35.*2.0-Lycm6.*Lzcm6.*dQ1.*dQ3.*m6.*t2.*t3.*t6.*t9.*t35.*2.0+Lycm6.*Lzcm6.*dQ1.*dQ4.*m6.*t2.*t4.*t6.*t8.*t35.*2.0+Lycm6.*Lzcm6.*dQ1.*dQ4.*m6.*t3.*t4.*t6.*t7.*t35.*2.0+Lycm6.*Lzcm6.*dQ1.*dQ2.*m6.*t2.*t8.*t10.*t11.*t34.*2.0+Lycm6.*Lzcm6.*dQ1.*dQ2.*m6.*t3.*t7.*t10.*t11.*t34.*2.0+Lycm6.*Lzcm6.*dQ1.*dQ2.*m6.*t6.*t7.*t8.*t9.*t35.*2.0+Lycm6.*Lzcm6.*dQ1.*dQ3.*m6.*t2.*t8.*t10.*t11.*t34.*2.0+Lycm6.*Lzcm6.*dQ1.*dQ3.*m6.*t3.*t7.*t10.*t11.*t34.*2.0+Lycm6.*Lzcm6.*dQ1.*dQ3.*m6.*t6.*t7.*t8.*t9.*t35.*2.0-Ixx6.*dQ1.*dQ2.*t2.*t3.*t5.*t6.*t9.*t10.*t11.*2.0-Ixx6.*dQ1.*dQ3.*t2.*t3.*t5.*t6.*t9.*t10.*t11.*2.0+Ixx6.*dQ1.*dQ2.*t5.*t6.*t7.*t8.*t9.*t10.*t11.*2.0+Ixx6.*dQ1.*dQ3.*t5.*t6.*t7.*t8.*t9.*t10.*t11.*2.0;
et572 = Ixx6.*dQ1.*dQ2.*t2.*t4.*t6.*t8.*t9.*t11.*t35.*-2.0-Ixx6.*dQ1.*dQ2.*t3.*t4.*t6.*t7.*t9.*t11.*t35.*2.0-Ixx6.*dQ1.*dQ3.*t2.*t4.*t6.*t8.*t9.*t11.*t35.*2.0-Ixx6.*dQ1.*dQ3.*t3.*t4.*t6.*t7.*t9.*t11.*t35.*2.0+Ixz6.*dQ1.*dQ2.*t2.*t4.*t5.*t8.*t9.*t10.*t11+Ixz6.*dQ1.*dQ2.*t3.*t4.*t5.*t7.*t9.*t10.*t11+Ixz6.*dQ1.*dQ3.*t2.*t4.*t5.*t8.*t9.*t10.*t11+Ixz6.*dQ1.*dQ3.*t3.*t4.*t5.*t7.*t9.*t10.*t11+Iyy6.*dQ1.*dQ2.*t2.*t3.*t5.*t6.*t9.*t10.*t11.*2.0+Iyy6.*dQ1.*dQ3.*t2.*t3.*t5.*t6.*t9.*t10.*t11.*2.0-Iyy6.*dQ1.*dQ2.*t5.*t6.*t7.*t8.*t9.*t10.*t11.*2.0-Iyy6.*dQ1.*dQ3.*t5.*t6.*t7.*t8.*t9.*t10.*t11.*2.0+Iyy6.*dQ1.*dQ2.*t2.*t4.*t6.*t8.*t9.*t11.*t35.*2.0+Iyy6.*dQ1.*dQ2.*t3.*t4.*t6.*t7.*t9.*t11.*t35.*2.0+Iyy6.*dQ1.*dQ3.*t2.*t4.*t6.*t8.*t9.*t11.*t35.*2.0+Iyy6.*dQ1.*dQ3.*t3.*t4.*t6.*t7.*t9.*t11.*t35.*2.0;
et573 = Iyz6.*dQ1.*dQ2.*t2.*t4.*t5.*t6.*t8.*t9.*t10+Iyz6.*dQ1.*dQ2.*t3.*t4.*t5.*t6.*t7.*t9.*t10+Iyz6.*dQ1.*dQ3.*t2.*t4.*t5.*t6.*t8.*t9.*t10+Iyz6.*dQ1.*dQ3.*t3.*t4.*t5.*t6.*t7.*t9.*t10+Izx6.*dQ1.*dQ2.*t2.*t4.*t5.*t8.*t9.*t10.*t11+Izx6.*dQ1.*dQ2.*t3.*t4.*t5.*t7.*t9.*t10.*t11+Izx6.*dQ1.*dQ3.*t2.*t4.*t5.*t8.*t9.*t10.*t11+Izx6.*dQ1.*dQ3.*t3.*t4.*t5.*t7.*t9.*t10.*t11+Izy6.*dQ1.*dQ2.*t2.*t4.*t5.*t6.*t8.*t9.*t10+Izy6.*dQ1.*dQ2.*t3.*t4.*t5.*t6.*t7.*t9.*t10+Izy6.*dQ1.*dQ3.*t2.*t4.*t5.*t6.*t8.*t9.*t10+Izy6.*dQ1.*dQ3.*t3.*t4.*t5.*t6.*t7.*t9.*t10+dQ1.*dQ2.*m6.*t2.*t4.*t6.*t8.*t9.*t11.*t17.*2.0+dQ1.*dQ2.*m6.*t3.*t4.*t6.*t7.*t9.*t11.*t17.*2.0+dQ1.*dQ3.*m6.*t2.*t4.*t6.*t8.*t9.*t11.*t17.*2.0+dQ1.*dQ3.*m6.*t3.*t4.*t6.*t7.*t9.*t11.*t17.*2.0-dQ1.*dQ2.*m6.*t2.*t4.*t6.*t8.*t9.*t11.*t20.*2.0;
et574 = dQ1.*dQ2.*m6.*t3.*t4.*t6.*t7.*t9.*t11.*t20.*-2.0-dQ1.*dQ3.*m6.*t2.*t4.*t6.*t8.*t9.*t11.*t20.*2.0-dQ1.*dQ3.*m6.*t3.*t4.*t6.*t7.*t9.*t11.*t20.*2.0+dQ1.*dQ2.*m6.*t2.*t3.*t5.*t6.*t9.*t10.*t11.*t17.*2.0+dQ1.*dQ3.*m6.*t2.*t3.*t5.*t6.*t9.*t10.*t11.*t17.*2.0-dQ1.*dQ4.*m6.*t2.*t4.*t5.*t6.*t8.*t10.*t11.*t17.*2.0-dQ1.*dQ4.*m6.*t3.*t4.*t5.*t6.*t7.*t10.*t11.*t17.*2.0-dQ1.*dQ2.*m6.*t2.*t3.*t5.*t6.*t9.*t10.*t11.*t20.*2.0-dQ1.*dQ3.*m6.*t2.*t3.*t5.*t6.*t9.*t10.*t11.*t20.*2.0+dQ1.*dQ4.*m6.*t2.*t4.*t5.*t6.*t8.*t10.*t11.*t20.*2.0+dQ1.*dQ4.*m6.*t3.*t4.*t5.*t6.*t7.*t10.*t11.*t20.*2.0-dQ1.*dQ2.*m6.*t5.*t6.*t7.*t8.*t9.*t10.*t11.*t17.*2.0-dQ1.*dQ3.*m6.*t5.*t6.*t7.*t8.*t9.*t10.*t11.*t17.*2.0+dQ1.*dQ2.*m6.*t5.*t6.*t7.*t8.*t9.*t10.*t11.*t20.*2.0;
et575 = dQ1.*dQ3.*m6.*t5.*t6.*t7.*t8.*t9.*t10.*t11.*t20.*2.0+dQ1.*dQ2.*m6.*t2.*t4.*t6.*t8.*t9.*t11.*t17.*t35.*2.0+dQ1.*dQ2.*m6.*t3.*t4.*t6.*t7.*t9.*t11.*t17.*t35.*2.0+dQ1.*dQ3.*m6.*t2.*t4.*t6.*t8.*t9.*t11.*t17.*t35.*2.0+dQ1.*dQ3.*m6.*t3.*t4.*t6.*t7.*t9.*t11.*t17.*t35.*2.0-dQ1.*dQ2.*m6.*t2.*t4.*t6.*t8.*t9.*t11.*t20.*t35.*2.0-dQ1.*dQ2.*m6.*t3.*t4.*t6.*t7.*t9.*t11.*t20.*t35.*2.0-dQ1.*dQ3.*m6.*t2.*t4.*t6.*t8.*t9.*t11.*t20.*t35.*2.0-dQ1.*dQ3.*m6.*t3.*t4.*t6.*t7.*t9.*t11.*t20.*t35.*2.0+Lxcm6.*Lycm6.*dQ1.*dQ2.*m6.*t2.*t3.*t4.*t6.*t10.*t11.*4.0+Lxcm6.*Lycm6.*dQ1.*dQ3.*m6.*t2.*t3.*t4.*t6.*t10.*t11.*4.0+Lxcm6.*Lycm6.*dQ1.*dQ5.*m6.*t2.*t4.*t5.*t6.*t8.*t11.*4.0+Lxcm6.*Lycm6.*dQ1.*dQ5.*m6.*t3.*t4.*t5.*t6.*t7.*t11.*4.0-Lxcm6.*Lycm6.*dQ1.*dQ2.*m6.*t4.*t6.*t7.*t8.*t10.*t11.*4.0;
et576 = Lxcm6.*Lycm6.*dQ1.*dQ3.*m6.*t4.*t6.*t7.*t8.*t10.*t11.*-4.0+Lxcm6.*Lycm6.*dQ1.*dQ2.*m6.*t2.*t3.*t5.*t9.*t10.*t36.*4.0+Lxcm6.*Lycm6.*dQ1.*dQ2.*m6.*t2.*t5.*t6.*t8.*t11.*t34.*8.0+Lxcm6.*Lycm6.*dQ1.*dQ2.*m6.*t3.*t5.*t6.*t7.*t11.*t34.*8.0+Lxcm6.*Lycm6.*dQ1.*dQ3.*m6.*t2.*t3.*t5.*t9.*t10.*t36.*4.0+Lxcm6.*Lycm6.*dQ1.*dQ3.*m6.*t2.*t5.*t6.*t8.*t11.*t34.*8.0+Lxcm6.*Lycm6.*dQ1.*dQ3.*m6.*t3.*t5.*t6.*t7.*t11.*t34.*8.0-Lxcm6.*Lycm6.*dQ1.*dQ4.*m6.*t2.*t4.*t5.*t8.*t10.*t36.*4.0-Lxcm6.*Lycm6.*dQ1.*dQ4.*m6.*t3.*t4.*t5.*t7.*t10.*t36.*4.0-Lxcm6.*Lycm6.*dQ1.*dQ2.*m6.*t5.*t7.*t8.*t9.*t10.*t36.*4.0-Lxcm6.*Lycm6.*dQ1.*dQ3.*m6.*t5.*t7.*t8.*t9.*t10.*t36.*4.0+Lxcm6.*Lycm6.*dQ1.*dQ2.*m6.*t2.*t4.*t8.*t9.*t35.*t36.*4.0+Lxcm6.*Lycm6.*dQ1.*dQ2.*m6.*t3.*t4.*t7.*t9.*t35.*t36.*4.0+Lxcm6.*Lycm6.*dQ1.*dQ3.*m6.*t2.*t4.*t8.*t9.*t35.*t36.*4.0;
et577 = Lxcm6.*Lycm6.*dQ1.*dQ3.*m6.*t3.*t4.*t7.*t9.*t35.*t36.*4.0+Lxcm6.*Lz5.*dQ1.*dQ2.*m6.*t2.*t4.*t5.*t8.*t9.*t10.*t11.*2.0+Lxcm6.*Lz5.*dQ1.*dQ2.*m6.*t3.*t4.*t5.*t7.*t9.*t10.*t11.*2.0+Lxcm6.*Lz5.*dQ1.*dQ3.*m6.*t2.*t4.*t5.*t8.*t9.*t10.*t11.*2.0+Lxcm6.*Lz5.*dQ1.*dQ3.*m6.*t3.*t4.*t5.*t7.*t9.*t10.*t11.*2.0+Lxcm6.*Lzcm6.*dQ1.*dQ2.*m6.*t2.*t4.*t5.*t8.*t9.*t10.*t11.*2.0+Lxcm6.*Lzcm6.*dQ1.*dQ2.*m6.*t3.*t4.*t5.*t7.*t9.*t10.*t11.*2.0+Lxcm6.*Lzcm6.*dQ1.*dQ3.*m6.*t2.*t4.*t5.*t8.*t9.*t10.*t11.*2.0+Lxcm6.*Lzcm6.*dQ1.*dQ3.*m6.*t3.*t4.*t5.*t7.*t9.*t10.*t11.*2.0+Lycm6.*Lz5.*dQ1.*dQ2.*m6.*t2.*t4.*t5.*t6.*t8.*t9.*t10.*2.0+Lycm6.*Lz5.*dQ1.*dQ2.*m6.*t3.*t4.*t5.*t6.*t7.*t9.*t10.*2.0+Lycm6.*Lz5.*dQ1.*dQ3.*m6.*t2.*t4.*t5.*t6.*t8.*t9.*t10.*2.0+Lycm6.*Lz5.*dQ1.*dQ3.*m6.*t3.*t4.*t5.*t6.*t7.*t9.*t10.*2.0+Lycm6.*Lzcm6.*dQ1.*dQ2.*m6.*t2.*t4.*t5.*t6.*t8.*t9.*t10.*2.0;
et578 = Lycm6.*Lzcm6.*dQ1.*dQ2.*m6.*t3.*t4.*t5.*t6.*t7.*t9.*t10.*2.0+Lycm6.*Lzcm6.*dQ1.*dQ3.*m6.*t2.*t4.*t5.*t6.*t8.*t9.*t10.*2.0+Lycm6.*Lzcm6.*dQ1.*dQ3.*m6.*t3.*t4.*t5.*t6.*t7.*t9.*t10.*2.0;
mt1 = [et370+et371;et372+et373+et374+et375+et376+et377+et378+et379+et380+et381+et382+et383+et384+et385+et386;et387+et388+et389+et390+et391+et392+et393+et394;et395+et396+et397+et398+et399+et400+et401+et402+et403+et404+et405+et406+et407+et408+et409+et410+et411+et412+et413+et414+et415+et416+et417+et418+et419+et420+et421+et422+et423+et424+et425+et426+et427+et428+et429+et430+et431+et432+et433+et434+et435+et436+et437+et438+et439+et440+et441+et442+et443+et444+et445+et446+et447+et448+et449+et450+et451+et452+et453+et454+et455+et456+et457+et458+et459+et460+et461+et462+et463+et464+et465+et466+et467+et468+et469+et470;et471+et472+et473+et474+et475+et476+et477+et478+et479+et480+et481+et482+et483+et484+et485+et486+et487+et488+et489+et490+et491+et492+et493+et494+et495+et496+et497+et498+et499+et500+et501+et502+et503+et504+et505+et506+et507+et508+et509+et510+et511+et512+et513+et514+et515+et516+et517+et518+et519+et520+et521+et522+et523+et524+et525+et526+et527+et528+et529+et530+et531+et532];
mt2 = [et533+et534+et535+et536+et537+et538+et539+et540+et541+et542+et543+et544+et545+et546+et547+et548+et549+et550+et551+et552+et553+et554+et555+et556+et557+et558+et559+et560+et561+et562+et563+et564+et565+et566+et567+et568+et569+et570+et571+et572+et573+et574+et575+et576+et577+et578];
out1 = [mt1;mt2];
end
